simulink model "mainModelDOEJF"  (R2025a)
settings: Solver=VariableStepAuto  StartTime=0  StopTime=1000  RelTol=1e-3
undefined symbols (not defined in the file): advectiveCoefficientScale, AmbientTemperature, coolantTempSourceTemperatureScale, massCoolantScale, massModuleScale, scaledAdvectiveCoefficient, scaledCoolantTemp, scaledMassCoolant, scaledMassModule
libraries: fl_lib x265, nesl_utility x68, coolantFlow_lib x65, thermalCoupledCellResolution_lib x32, heatGenerationForCellResolvedModel x32, batt_lib x1, coolantFlowSwitch_lib x1
(part 3 of 4)

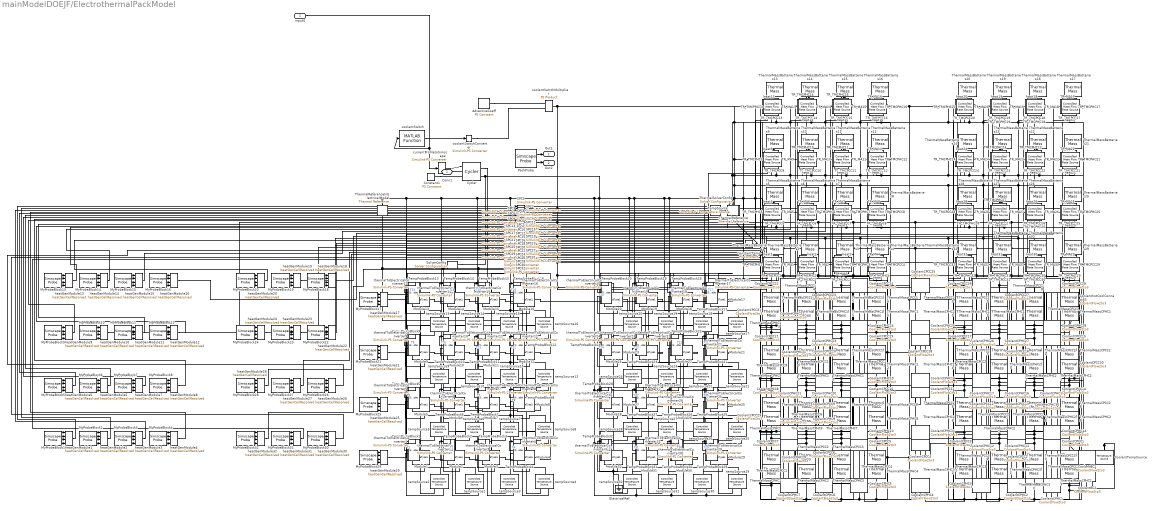
== system mainModelDOEJF/ElectrothermalPackModel ==
  input0 : Inport
  AdvectiveCoeff : fl_lib/Physical Signals/Sources/PS Constant  constant=advectiveCoefficientScale * scaledAdvectiveCoefficient W/K
  Constant1 : fl_lib/Physical Signals/Sources/PS Constant  constant=1
  ConstantTemp : fl_lib/Physical Signals/Sources/PS Constant  constant=AmbientTemperature
  CoolantBC1 : coolantFlow_lib/CoolantFlow2to3  SystemSampleTime=-1  VariantActivationTime=update diagram  EmptyChoice=off  PassThrough=off  PassThroughVariantControl=(default)  EmptyChoiceVariantControl=(default)  AllowFlexibleInterface=on  Latency=0  AutoFrameSizeCalculation=off
  CoolantBC2 : coolantFlow_lib/CoolantFlow2to3  SystemSampleTime=-1  VariantActivationTime=update diagram  EmptyChoice=off  PassThrough=off  PassThroughVariantControl=(default)  EmptyChoiceVariantControl=(default)  AllowFlexibleInterface=on  Latency=0  AutoFrameSizeCalculation=off
  CoolantCPCC{1..31} (31 alike) : coolantFlow_lib/CoolantFlow2to3  SystemSampleTime=-1  VariantActivationTime=update diagram  EmptyChoice=off  PassThrough=off  PassThroughVariantControl=(default)  EmptyChoiceVariantControl=(default)  AllowFlexibleInterface=on  Latency=0  AutoFrameSizeCalculation=off
  CoolantCPHC{1..31} (31 alike) : coolantFlow_lib/CoolantFlow2to3  SystemSampleTime=-1  VariantActivationTime=update diagram  EmptyChoice=off  PassThrough=off  PassThroughVariantControl=(default)  EmptyChoiceVariantControl=(default)  AllowFlexibleInterface=on  Latency=0  AutoFrameSizeCalculation=off
  CoolantTempSource : fl_lib/Thermal/Thermal Sources/Temperature Source  temperature=coolantTempSourceTemperatureScale * scaledCoolantTemp K
  CoolanthotCoolConnect63 : coolantFlow_lib/CoolantFlow2to3  SystemSampleTime=-1  VariantActivationTime=update diagram  EmptyChoice=off  PassThrough=off  PassThroughVariantControl=(default)  EmptyChoiceVariantControl=(default)  AllowFlexibleInterface=on  Latency=0  AutoFrameSizeCalculation=off
  Cycler : batt_lib/Cyclers/Cycler  current_option=simscape.battery.enum.cyclers.positive_current.Discharge  configuration_option=simscape.battery.enum.cyclers.device_configuration.Cycler
      settings: InternalSimscapePortConfiguration="{\"Bottom\":[],\"Left\":[{\"id\":\"iT\",\"label\":\"i\",\"type\":\"input\"},{\"id\":\"vT\",\"label\":\"v\",\"type\":\"input\"},{\"id\":\"c\",\"label\":\"c\",\"type\":\"input\"}],\"Right\":[{\"id\":\"p\",\"label\":\"+\",\"type\":\"foundation.electrical.electrical\"},{\"id\":\"n\",\"label\":\"-\",\"type\":\"foundation.electrical.electrical\"}],\"Top\":[]}"
  ElectricalRef : fl_lib/Electrical/Electrical Elements/Electrical Reference
  Module1 : thermalCoupledCellResolution_lib/Modules/ModuleType1  BatteryCapacityCell=Module01.BatteryCapacityCell A*hr  BatteryCapacityCellPercentDeviation=Module01.BatteryCapacityCellPercentDeviation  ExtrapolationMethodCell=simscape.enum.extrapolation.nearest  SOCBreakpointsCell=Module01.SOCBreakpointsCell  SOCBreakpointsCellPercentDeviation=Module01.SOCBreakpointsCellPercentDeviation  TemperatureBreakpointsCell=Module01.TemperatureBreakpointsCell K  TemperatureBreakpointsCellPercentDeviation=Module01.TemperatureBreakpointsCellPercentDeviation  OpenCircuitVoltageThermalCell=Module01.OpenCircuitVoltageThermalCell V  OpenCircuitVoltageThermalCellPercentDeviation=Module01.OpenCircuitVoltageThermalCellPercentDeviation  VoltageRangeCell=Module01.VoltageRangeCell V  VoltageRangeCellPercentDeviation=Module01.VoltageRangeCellPercentDeviation  ResistanceSOCBreakpointsCell=Module01.ResistanceSOCBreakpointsCell  ResistanceSOCBreakpointsCellPercentDeviation=Module01.ResistanceSOCBreakpointsCellPercentDeviation  ResistanceTemperatureBreakpointsCell=Module01.ResistanceTemperatureBreakpointsCell K  ResistanceTemperatureBreakpointsCellPercentDeviation=Module01.ResistanceTemperatureBreakpointsCellPercentDeviation  R0ThermalCell=Module01.R0ThermalCell Ohm  R0ThermalCellPercentDeviation=Module01.R0ThermalCellPercentDeviation  R1ThermalCell=Module01.R1ThermalCell Ohm  R1ThermalCellPercentDeviation=Module01.R1ThermalCellPercentDeviation  Tau1ThermalCell=Module01.Tau1ThermalCell s  Tau1ThermalCellPercentDeviation=Module01.Tau1ThermalCellPercentDeviation  BatteryThermalMassCell=Module01.BatteryThermalMassCell J/K  BatteryThermalMassCellPercentDeviation=Module01.BatteryThermalMassCellPercentDeviation  AmbientResistance=Module01.AmbientResistance K/W  P=2  S=6  socCell_specify=on  socCell_priority=High  socCell=Module01.socCell  socCell_nominal_specify=off  socCell_nominal_value=1  socCell_nominal_unit=1  batteryVoltage_specify=on  batteryVoltage_priority=None  batteryVoltage=Module01.batteryVoltage V  batteryVoltage_nominal_specify=off  batteryVoltage_nominal_value=1  batteryVoltage_nominal_unit=V  batteryCurrent_specify=on  batteryCurrent_priority=None  batteryCurrent=Module01.batteryCurrent A  batteryCurrent_nominal_specify=off  batteryCurrent_nominal_value=1  batteryCurrent_nominal_unit=A  numCycles_specify=on  numCycles_priority=High  numCycles=Module01.numCycles  numCycles_nominal_specify=off  numCycles_nominal_value=1  numCycles_nominal_unit=1  batteryTemperature_specify=on  batteryTemperature_priority=High  batteryTemperature=Module01.batteryTemperature K  batteryTemperature_nominal_specify=off  batteryTemperature_nominal_value=1  batteryTemperature_nominal_unit=K  vParallelAssembly_specify=on  vParallelAssembly_priority=None  vParallelAssembly=Module01.vParallelAssembly V  vParallelAssembly_nominal_specify=off  vParallelAssembly_nominal_value=1  vParallelAssembly_nominal_unit=V  socParallelAssembly_specify=on  socParallelAssembly_priority=None  socParallelAssembly=Module01.socParallelAssembly  socParallelAssembly_nominal_specify=off  socParallelAssembly_nominal_value=1  socParallelAssembly_nominal_unit=1
      settings: InternalSimscapePortConfiguration="{\"Bottom\":[{\"id\":\"n\",\"label\":\"-\",\"type\":\"foundation.electrical.electrical\"}],\"Left\":[{\"id\":\"AmbH\",\"label\":\"AmbH\",\"type\":\"foundation.thermal.thermal\"}],\"Right\":[],\"Top\":[{\"id\":\"p\",\"label\":\"+\",\"type\":\"foundation.electrical.electrical\"}]}"
  Module10 : thermalCoupledCellResolution_lib/Modules/ModuleType1  BatteryCapacityCell=Module10.BatteryCapacityCell A*hr  BatteryCapacityCellPercentDeviation=Module10.BatteryCapacityCellPercentDeviation  ExtrapolationMethodCell=simscape.enum.extrapolation.nearest  SOCBreakpointsCell=Module10.SOCBreakpointsCell  SOCBreakpointsCellPercentDeviation=Module10.SOCBreakpointsCellPercentDeviation  TemperatureBreakpointsCell=Module10.TemperatureBreakpointsCell K  TemperatureBreakpointsCellPercentDeviation=Module10.TemperatureBreakpointsCellPercentDeviation  OpenCircuitVoltageThermalCell=Module10.OpenCircuitVoltageThermalCell V  OpenCircuitVoltageThermalCellPercentDeviation=Module10.OpenCircuitVoltageThermalCellPercentDeviation  VoltageRangeCell=Module10.VoltageRangeCell V  VoltageRangeCellPercentDeviation=Module10.VoltageRangeCellPercentDeviation  ResistanceSOCBreakpointsCell=Module10.ResistanceSOCBreakpointsCell  ResistanceSOCBreakpointsCellPercentDeviation=Module10.ResistanceSOCBreakpointsCellPercentDeviation  ResistanceTemperatureBreakpointsCell=Module10.ResistanceTemperatureBreakpointsCell K  ResistanceTemperatureBreakpointsCellPercentDeviation=Module10.ResistanceTemperatureBreakpointsCellPercentDeviation  R0ThermalCell=Module10.R0ThermalCell Ohm  R0ThermalCellPercentDeviation=Module10.R0ThermalCellPercentDeviation  R1ThermalCell=Module10.R1ThermalCell Ohm  R1ThermalCellPercentDeviation=Module10.R1ThermalCellPercentDeviation  Tau1ThermalCell=Module10.Tau1ThermalCell s  Tau1ThermalCellPercentDeviation=Module10.Tau1ThermalCellPercentDeviation  BatteryThermalMassCell=Module10.BatteryThermalMassCell J/K  BatteryThermalMassCellPercentDeviation=Module10.BatteryThermalMassCellPercentDeviation  AmbientResistance=Module10.AmbientResistance K/W  P=2  S=6  socCell_specify=on  socCell_priority=High  socCell=Module10.socCell  socCell_nominal_specify=off  socCell_nominal_value=1  socCell_nominal_unit=1  batteryVoltage_specify=on  batteryVoltage_priority=None  batteryVoltage=Module10.batteryVoltage V  batteryVoltage_nominal_specify=off  batteryVoltage_nominal_value=1  batteryVoltage_nominal_unit=V  batteryCurrent_specify=on  batteryCurrent_priority=None  batteryCurrent=Module10.batteryCurrent A  batteryCurrent_nominal_specify=off  batteryCurrent_nominal_value=1  batteryCurrent_nominal_unit=A  numCycles_specify=on  numCycles_priority=High  numCycles=Module10.numCycles  numCycles_nominal_specify=off  numCycles_nominal_value=1  numCycles_nominal_unit=1  batteryTemperature_specify=on  batteryTemperature_priority=High  batteryTemperature=Module10.batteryTemperature K  batteryTemperature_nominal_specify=off  batteryTemperature_nominal_value=1  batteryTemperature_nominal_unit=K  vParallelAssembly_specify=on  vParallelAssembly_priority=None  vParallelAssembly=Module10.vParallelAssembly V  vParallelAssembly_nominal_specify=off  vParallelAssembly_nominal_value=1  vParallelAssembly_nominal_unit=V  socParallelAssembly_specify=on  socParallelAssembly_priority=None  socParallelAssembly=Module10.socParallelAssembly  socParallelAssembly_nominal_specify=off  socParallelAssembly_nominal_value=1  socParallelAssembly_nominal_unit=1
      settings: InternalSimscapePortConfiguration="{\"Bottom\":[{\"id\":\"n\",\"label\":\"-\",\"type\":\"foundation.electrical.electrical\"}],\"Left\":[{\"id\":\"AmbH\",\"label\":\"AmbH\",\"type\":\"foundation.thermal.thermal\"}],\"Right\":[],\"Top\":[{\"id\":\"p\",\"label\":\"+\",\"type\":\"foundation.electrical.electrical\"}]}"
  Module11 : thermalCoupledCellResolution_lib/Modules/ModuleType1  BatteryCapacityCell=Module11.BatteryCapacityCell A*hr  BatteryCapacityCellPercentDeviation=Module11.BatteryCapacityCellPercentDeviation  ExtrapolationMethodCell=simscape.enum.extrapolation.nearest  SOCBreakpointsCell=Module11.SOCBreakpointsCell  SOCBreakpointsCellPercentDeviation=Module11.SOCBreakpointsCellPercentDeviation  TemperatureBreakpointsCell=Module11.TemperatureBreakpointsCell K  TemperatureBreakpointsCellPercentDeviation=Module11.TemperatureBreakpointsCellPercentDeviation  OpenCircuitVoltageThermalCell=Module11.OpenCircuitVoltageThermalCell V  OpenCircuitVoltageThermalCellPercentDeviation=Module11.OpenCircuitVoltageThermalCellPercentDeviation  VoltageRangeCell=Module11.VoltageRangeCell V  VoltageRangeCellPercentDeviation=Module11.VoltageRangeCellPercentDeviation  ResistanceSOCBreakpointsCell=Module11.ResistanceSOCBreakpointsCell  ResistanceSOCBreakpointsCellPercentDeviation=Module11.ResistanceSOCBreakpointsCellPercentDeviation  ResistanceTemperatureBreakpointsCell=Module11.ResistanceTemperatureBreakpointsCell K  ResistanceTemperatureBreakpointsCellPercentDeviation=Module11.ResistanceTemperatureBreakpointsCellPercentDeviation  R0ThermalCell=Module11.R0ThermalCell Ohm  R0ThermalCellPercentDeviation=Module11.R0ThermalCellPercentDeviation  R1ThermalCell=Module11.R1ThermalCell Ohm  R1ThermalCellPercentDeviation=Module11.R1ThermalCellPercentDeviation  Tau1ThermalCell=Module11.Tau1ThermalCell s  Tau1ThermalCellPercentDeviation=Module11.Tau1ThermalCellPercentDeviation  BatteryThermalMassCell=Module11.BatteryThermalMassCell J/K  BatteryThermalMassCellPercentDeviation=Module11.BatteryThermalMassCellPercentDeviation  AmbientResistance=Module11.AmbientResistance K/W  P=2  S=6  socCell_specify=on  socCell_priority=High  socCell=Module11.socCell  socCell_nominal_specify=off  socCell_nominal_value=1  socCell_nominal_unit=1  batteryVoltage_specify=on  batteryVoltage_priority=None  batteryVoltage=Module11.batteryVoltage V  batteryVoltage_nominal_specify=off  batteryVoltage_nominal_value=1  batteryVoltage_nominal_unit=V  batteryCurrent_specify=on  batteryCurrent_priority=None  batteryCurrent=Module11.batteryCurrent A  batteryCurrent_nominal_specify=off  batteryCurrent_nominal_value=1  batteryCurrent_nominal_unit=A  numCycles_specify=on  numCycles_priority=High  numCycles=Module11.numCycles  numCycles_nominal_specify=off  numCycles_nominal_value=1  numCycles_nominal_unit=1  batteryTemperature_specify=on  batteryTemperature_priority=High  batteryTemperature=Module11.batteryTemperature K  batteryTemperature_nominal_specify=off  batteryTemperature_nominal_value=1  batteryTemperature_nominal_unit=K  vParallelAssembly_specify=on  vParallelAssembly_priority=None  vParallelAssembly=Module11.vParallelAssembly V  vParallelAssembly_nominal_specify=off  vParallelAssembly_nominal_value=1  vParallelAssembly_nominal_unit=V  socParallelAssembly_specify=on  socParallelAssembly_priority=None  socParallelAssembly=Module11.socParallelAssembly  socParallelAssembly_nominal_specify=off  socParallelAssembly_nominal_value=1  socParallelAssembly_nominal_unit=1
      settings: InternalSimscapePortConfiguration="{\"Bottom\":[{\"id\":\"n\",\"label\":\"-\",\"type\":\"foundation.electrical.electrical\"}],\"Left\":[{\"id\":\"AmbH\",\"label\":\"AmbH\",\"type\":\"foundation.thermal.thermal\"}],\"Right\":[],\"Top\":[{\"id\":\"p\",\"label\":\"+\",\"type\":\"foundation.electrical.electrical\"}]}"
  Module12 : thermalCoupledCellResolution_lib/Modules/ModuleType1  BatteryCapacityCell=Module12.BatteryCapacityCell A*hr  BatteryCapacityCellPercentDeviation=Module12.BatteryCapacityCellPercentDeviation  ExtrapolationMethodCell=simscape.enum.extrapolation.nearest  SOCBreakpointsCell=Module12.SOCBreakpointsCell  SOCBreakpointsCellPercentDeviation=Module12.SOCBreakpointsCellPercentDeviation  TemperatureBreakpointsCell=Module12.TemperatureBreakpointsCell K  TemperatureBreakpointsCellPercentDeviation=Module12.TemperatureBreakpointsCellPercentDeviation  OpenCircuitVoltageThermalCell=Module12.OpenCircuitVoltageThermalCell V  OpenCircuitVoltageThermalCellPercentDeviation=Module12.OpenCircuitVoltageThermalCellPercentDeviation  VoltageRangeCell=Module12.VoltageRangeCell V  VoltageRangeCellPercentDeviation=Module12.VoltageRangeCellPercentDeviation  ResistanceSOCBreakpointsCell=Module12.ResistanceSOCBreakpointsCell  ResistanceSOCBreakpointsCellPercentDeviation=Module12.ResistanceSOCBreakpointsCellPercentDeviation  ResistanceTemperatureBreakpointsCell=Module12.ResistanceTemperatureBreakpointsCell K  ResistanceTemperatureBreakpointsCellPercentDeviation=Module12.ResistanceTemperatureBreakpointsCellPercentDeviation  R0ThermalCell=Module12.R0ThermalCell Ohm  R0ThermalCellPercentDeviation=Module12.R0ThermalCellPercentDeviation  R1ThermalCell=Module12.R1ThermalCell Ohm  R1ThermalCellPercentDeviation=Module12.R1ThermalCellPercentDeviation  Tau1ThermalCell=Module12.Tau1ThermalCell s  Tau1ThermalCellPercentDeviation=Module12.Tau1ThermalCellPercentDeviation  BatteryThermalMassCell=Module12.BatteryThermalMassCell J/K  BatteryThermalMassCellPercentDeviation=Module12.BatteryThermalMassCellPercentDeviation  AmbientResistance=Module12.AmbientResistance K/W  P=2  S=6  socCell_specify=on  socCell_priority=High  socCell=Module12.socCell  socCell_nominal_specify=off  socCell_nominal_value=1  socCell_nominal_unit=1  batteryVoltage_specify=on  batteryVoltage_priority=None  batteryVoltage=Module12.batteryVoltage V  batteryVoltage_nominal_specify=off  batteryVoltage_nominal_value=1  batteryVoltage_nominal_unit=V  batteryCurrent_specify=on  batteryCurrent_priority=None  batteryCurrent=Module12.batteryCurrent A  batteryCurrent_nominal_specify=off  batteryCurrent_nominal_value=1  batteryCurrent_nominal_unit=A  numCycles_specify=on  numCycles_priority=High  numCycles=Module12.numCycles  numCycles_nominal_specify=off  numCycles_nominal_value=1  numCycles_nominal_unit=1  batteryTemperature_specify=on  batteryTemperature_priority=High  batteryTemperature=Module12.batteryTemperature K  batteryTemperature_nominal_specify=off  batteryTemperature_nominal_value=1  batteryTemperature_nominal_unit=K  vParallelAssembly_specify=on  vParallelAssembly_priority=None  vParallelAssembly=Module12.vParallelAssembly V  vParallelAssembly_nominal_specify=off  vParallelAssembly_nominal_value=1  vParallelAssembly_nominal_unit=V  socParallelAssembly_specify=on  socParallelAssembly_priority=None  socParallelAssembly=Module12.socParallelAssembly  socParallelAssembly_nominal_specify=off  socParallelAssembly_nominal_value=1  socParallelAssembly_nominal_unit=1
      settings: InternalSimscapePortConfiguration="{\"Bottom\":[{\"id\":\"n\",\"label\":\"-\",\"type\":\"foundation.electrical.electrical\"}],\"Left\":[{\"id\":\"AmbH\",\"label\":\"AmbH\",\"type\":\"foundation.thermal.thermal\"}],\"Right\":[],\"Top\":[{\"id\":\"p\",\"label\":\"+\",\"type\":\"foundation.electrical.electrical\"}]}"
  Module13 : thermalCoupledCellResolution_lib/Modules/ModuleType1  BatteryCapacityCell=Module13.BatteryCapacityCell A*hr  BatteryCapacityCellPercentDeviation=Module13.BatteryCapacityCellPercentDeviation  ExtrapolationMethodCell=simscape.enum.extrapolation.nearest  SOCBreakpointsCell=Module13.SOCBreakpointsCell  SOCBreakpointsCellPercentDeviation=Module13.SOCBreakpointsCellPercentDeviation  TemperatureBreakpointsCell=Module13.TemperatureBreakpointsCell K  TemperatureBreakpointsCellPercentDeviation=Module13.TemperatureBreakpointsCellPercentDeviation  OpenCircuitVoltageThermalCell=Module13.OpenCircuitVoltageThermalCell V  OpenCircuitVoltageThermalCellPercentDeviation=Module13.OpenCircuitVoltageThermalCellPercentDeviation  VoltageRangeCell=Module13.VoltageRangeCell V  VoltageRangeCellPercentDeviation=Module13.VoltageRangeCellPercentDeviation  ResistanceSOCBreakpointsCell=Module13.ResistanceSOCBreakpointsCell  ResistanceSOCBreakpointsCellPercentDeviation=Module13.ResistanceSOCBreakpointsCellPercentDeviation  ResistanceTemperatureBreakpointsCell=Module13.ResistanceTemperatureBreakpointsCell K  ResistanceTemperatureBreakpointsCellPercentDeviation=Module13.ResistanceTemperatureBreakpointsCellPercentDeviation  R0ThermalCell=Module13.R0ThermalCell Ohm  R0ThermalCellPercentDeviation=Module13.R0ThermalCellPercentDeviation  R1ThermalCell=Module13.R1ThermalCell Ohm  R1ThermalCellPercentDeviation=Module13.R1ThermalCellPercentDeviation  Tau1ThermalCell=Module13.Tau1ThermalCell s  Tau1ThermalCellPercentDeviation=Module13.Tau1ThermalCellPercentDeviation  BatteryThermalMassCell=Module13.BatteryThermalMassCell J/K  BatteryThermalMassCellPercentDeviation=Module13.BatteryThermalMassCellPercentDeviation  AmbientResistance=Module13.AmbientResistance K/W  P=2  S=6  socCell_specify=on  socCell_priority=High  socCell=Module13.socCell  socCell_nominal_specify=off  socCell_nominal_value=1  socCell_nominal_unit=1  batteryVoltage_specify=on  batteryVoltage_priority=None  batteryVoltage=Module13.batteryVoltage V  batteryVoltage_nominal_specify=off  batteryVoltage_nominal_value=1  batteryVoltage_nominal_unit=V  batteryCurrent_specify=on  batteryCurrent_priority=None  batteryCurrent=Module13.batteryCurrent A  batteryCurrent_nominal_specify=off  batteryCurrent_nominal_value=1  batteryCurrent_nominal_unit=A  numCycles_specify=on  numCycles_priority=High  numCycles=Module13.numCycles  numCycles_nominal_specify=off  numCycles_nominal_value=1  numCycles_nominal_unit=1  batteryTemperature_specify=on  batteryTemperature_priority=High  batteryTemperature=Module13.batteryTemperature K  batteryTemperature_nominal_specify=off  batteryTemperature_nominal_value=1  batteryTemperature_nominal_unit=K  vParallelAssembly_specify=on  vParallelAssembly_priority=None  vParallelAssembly=Module13.vParallelAssembly V  vParallelAssembly_nominal_specify=off  vParallelAssembly_nominal_value=1  vParallelAssembly_nominal_unit=V  socParallelAssembly_specify=on  socParallelAssembly_priority=None  socParallelAssembly=Module13.socParallelAssembly  socParallelAssembly_nominal_specify=off  socParallelAssembly_nominal_value=1  socParallelAssembly_nominal_unit=1
      settings: InternalSimscapePortConfiguration="{\"Bottom\":[{\"id\":\"n\",\"label\":\"-\",\"type\":\"foundation.electrical.electrical\"}],\"Left\":[{\"id\":\"AmbH\",\"label\":\"AmbH\",\"type\":\"foundation.thermal.thermal\"}],\"Right\":[],\"Top\":[{\"id\":\"p\",\"label\":\"+\",\"type\":\"foundation.electrical.electrical\"}]}"
  Module14 : thermalCoupledCellResolution_lib/Modules/ModuleType1  BatteryCapacityCell=Module14.BatteryCapacityCell A*hr  BatteryCapacityCellPercentDeviation=Module14.BatteryCapacityCellPercentDeviation  ExtrapolationMethodCell=simscape.enum.extrapolation.nearest  SOCBreakpointsCell=Module14.SOCBreakpointsCell  SOCBreakpointsCellPercentDeviation=Module14.SOCBreakpointsCellPercentDeviation  TemperatureBreakpointsCell=Module14.TemperatureBreakpointsCell K  TemperatureBreakpointsCellPercentDeviation=Module14.TemperatureBreakpointsCellPercentDeviation  OpenCircuitVoltageThermalCell=Module14.OpenCircuitVoltageThermalCell V  OpenCircuitVoltageThermalCellPercentDeviation=Module14.OpenCircuitVoltageThermalCellPercentDeviation  VoltageRangeCell=Module14.VoltageRangeCell V  VoltageRangeCellPercentDeviation=Module14.VoltageRangeCellPercentDeviation  ResistanceSOCBreakpointsCell=Module14.ResistanceSOCBreakpointsCell  ResistanceSOCBreakpointsCellPercentDeviation=Module14.ResistanceSOCBreakpointsCellPercentDeviation  ResistanceTemperatureBreakpointsCell=Module14.ResistanceTemperatureBreakpointsCell K  ResistanceTemperatureBreakpointsCellPercentDeviation=Module14.ResistanceTemperatureBreakpointsCellPercentDeviation  R0ThermalCell=Module14.R0ThermalCell Ohm  R0ThermalCellPercentDeviation=Module14.R0ThermalCellPercentDeviation  R1ThermalCell=Module14.R1ThermalCell Ohm  R1ThermalCellPercentDeviation=Module14.R1ThermalCellPercentDeviation  Tau1ThermalCell=Module14.Tau1ThermalCell s  Tau1ThermalCellPercentDeviation=Module14.Tau1ThermalCellPercentDeviation  BatteryThermalMassCell=Module14.BatteryThermalMassCell J/K  BatteryThermalMassCellPercentDeviation=Module14.BatteryThermalMassCellPercentDeviation  AmbientResistance=Module14.AmbientResistance K/W  P=2  S=6  socCell_specify=on  socCell_priority=High  socCell=Module14.socCell  socCell_nominal_specify=off  socCell_nominal_value=1  socCell_nominal_unit=1  batteryVoltage_specify=on  batteryVoltage_priority=None  batteryVoltage=Module14.batteryVoltage V  batteryVoltage_nominal_specify=off  batteryVoltage_nominal_value=1  batteryVoltage_nominal_unit=V  batteryCurrent_specify=on  batteryCurrent_priority=None  batteryCurrent=Module14.batteryCurrent A  batteryCurrent_nominal_specify=off  batteryCurrent_nominal_value=1  batteryCurrent_nominal_unit=A  numCycles_specify=on  numCycles_priority=High  numCycles=Module14.numCycles  numCycles_nominal_specify=off  numCycles_nominal_value=1  numCycles_nominal_unit=1  batteryTemperature_specify=on  batteryTemperature_priority=High  batteryTemperature=Module14.batteryTemperature K  batteryTemperature_nominal_specify=off  batteryTemperature_nominal_value=1  batteryTemperature_nominal_unit=K  vParallelAssembly_specify=on  vParallelAssembly_priority=None  vParallelAssembly=Module14.vParallelAssembly V  vParallelAssembly_nominal_specify=off  vParallelAssembly_nominal_value=1  vParallelAssembly_nominal_unit=V  socParallelAssembly_specify=on  socParallelAssembly_priority=None  socParallelAssembly=Module14.socParallelAssembly  socParallelAssembly_nominal_specify=off  socParallelAssembly_nominal_value=1  socParallelAssembly_nominal_unit=1
      settings: InternalSimscapePortConfiguration="{\"Bottom\":[{\"id\":\"n\",\"label\":\"-\",\"type\":\"foundation.electrical.electrical\"}],\"Left\":[{\"id\":\"AmbH\",\"label\":\"AmbH\",\"type\":\"foundation.thermal.thermal\"}],\"Right\":[],\"Top\":[{\"id\":\"p\",\"label\":\"+\",\"type\":\"foundation.electrical.electrical\"}]}"
  Module15 : thermalCoupledCellResolution_lib/Modules/ModuleType1  BatteryCapacityCell=Module15.BatteryCapacityCell A*hr  BatteryCapacityCellPercentDeviation=Module15.BatteryCapacityCellPercentDeviation  ExtrapolationMethodCell=simscape.enum.extrapolation.nearest  SOCBreakpointsCell=Module15.SOCBreakpointsCell  SOCBreakpointsCellPercentDeviation=Module15.SOCBreakpointsCellPercentDeviation  TemperatureBreakpointsCell=Module15.TemperatureBreakpointsCell K  TemperatureBreakpointsCellPercentDeviation=Module15.TemperatureBreakpointsCellPercentDeviation  OpenCircuitVoltageThermalCell=Module15.OpenCircuitVoltageThermalCell V  OpenCircuitVoltageThermalCellPercentDeviation=Module15.OpenCircuitVoltageThermalCellPercentDeviation  VoltageRangeCell=Module15.VoltageRangeCell V  VoltageRangeCellPercentDeviation=Module15.VoltageRangeCellPercentDeviation  ResistanceSOCBreakpointsCell=Module15.ResistanceSOCBreakpointsCell  ResistanceSOCBreakpointsCellPercentDeviation=Module15.ResistanceSOCBreakpointsCellPercentDeviation  ResistanceTemperatureBreakpointsCell=Module15.ResistanceTemperatureBreakpointsCell K  ResistanceTemperatureBreakpointsCellPercentDeviation=Module15.ResistanceTemperatureBreakpointsCellPercentDeviation  R0ThermalCell=Module15.R0ThermalCell Ohm  R0ThermalCellPercentDeviation=Module15.R0ThermalCellPercentDeviation  R1ThermalCell=Module15.R1ThermalCell Ohm  R1ThermalCellPercentDeviation=Module15.R1ThermalCellPercentDeviation  Tau1ThermalCell=Module15.Tau1ThermalCell s  Tau1ThermalCellPercentDeviation=Module15.Tau1ThermalCellPercentDeviation  BatteryThermalMassCell=Module15.BatteryThermalMassCell J/K  BatteryThermalMassCellPercentDeviation=Module15.BatteryThermalMassCellPercentDeviation  AmbientResistance=Module15.AmbientResistance K/W  P=2  S=6  socCell_specify=on  socCell_priority=High  socCell=Module15.socCell  socCell_nominal_specify=off  socCell_nominal_value=1  socCell_nominal_unit=1  batteryVoltage_specify=on  batteryVoltage_priority=None  batteryVoltage=Module15.batteryVoltage V  batteryVoltage_nominal_specify=off  batteryVoltage_nominal_value=1  batteryVoltage_nominal_unit=V  batteryCurrent_specify=on  batteryCurrent_priority=None  batteryCurrent=Module15.batteryCurrent A  batteryCurrent_nominal_specify=off  batteryCurrent_nominal_value=1  batteryCurrent_nominal_unit=A  numCycles_specify=on  numCycles_priority=High  numCycles=Module15.numCycles  numCycles_nominal_specify=off  numCycles_nominal_value=1  numCycles_nominal_unit=1  batteryTemperature_specify=on  batteryTemperature_priority=High  batteryTemperature=Module15.batteryTemperature K  batteryTemperature_nominal_specify=off  batteryTemperature_nominal_value=1  batteryTemperature_nominal_unit=K  vParallelAssembly_specify=on  vParallelAssembly_priority=None  vParallelAssembly=Module15.vParallelAssembly V  vParallelAssembly_nominal_specify=off  vParallelAssembly_nominal_value=1  vParallelAssembly_nominal_unit=V  socParallelAssembly_specify=on  socParallelAssembly_priority=None  socParallelAssembly=Module15.socParallelAssembly  socParallelAssembly_nominal_specify=off  socParallelAssembly_nominal_value=1  socParallelAssembly_nominal_unit=1
      settings: InternalSimscapePortConfiguration="{\"Bottom\":[{\"id\":\"n\",\"label\":\"-\",\"type\":\"foundation.electrical.electrical\"}],\"Left\":[{\"id\":\"AmbH\",\"label\":\"AmbH\",\"type\":\"foundation.thermal.thermal\"}],\"Right\":[],\"Top\":[{\"id\":\"p\",\"label\":\"+\",\"type\":\"foundation.electrical.electrical\"}]}"
  Module16 : thermalCoupledCellResolution_lib/Modules/ModuleType1  BatteryCapacityCell=Module16.BatteryCapacityCell A*hr  BatteryCapacityCellPercentDeviation=Module16.BatteryCapacityCellPercentDeviation  ExtrapolationMethodCell=simscape.enum.extrapolation.nearest  SOCBreakpointsCell=Module16.SOCBreakpointsCell  SOCBreakpointsCellPercentDeviation=Module16.SOCBreakpointsCellPercentDeviation  TemperatureBreakpointsCell=Module16.TemperatureBreakpointsCell K  TemperatureBreakpointsCellPercentDeviation=Module16.TemperatureBreakpointsCellPercentDeviation  OpenCircuitVoltageThermalCell=Module16.OpenCircuitVoltageThermalCell V  OpenCircuitVoltageThermalCellPercentDeviation=Module16.OpenCircuitVoltageThermalCellPercentDeviation  VoltageRangeCell=Module16.VoltageRangeCell V  VoltageRangeCellPercentDeviation=Module16.VoltageRangeCellPercentDeviation  ResistanceSOCBreakpointsCell=Module16.ResistanceSOCBreakpointsCell  ResistanceSOCBreakpointsCellPercentDeviation=Module16.ResistanceSOCBreakpointsCellPercentDeviation  ResistanceTemperatureBreakpointsCell=Module16.ResistanceTemperatureBreakpointsCell K  ResistanceTemperatureBreakpointsCellPercentDeviation=Module16.ResistanceTemperatureBreakpointsCellPercentDeviation  R0ThermalCell=Module16.R0ThermalCell Ohm  R0ThermalCellPercentDeviation=Module16.R0ThermalCellPercentDeviation  R1ThermalCell=Module16.R1ThermalCell Ohm  R1ThermalCellPercentDeviation=Module16.R1ThermalCellPercentDeviation  Tau1ThermalCell=Module16.Tau1ThermalCell s  Tau1ThermalCellPercentDeviation=Module16.Tau1ThermalCellPercentDeviation  BatteryThermalMassCell=Module16.BatteryThermalMassCell J/K  BatteryThermalMassCellPercentDeviation=Module16.BatteryThermalMassCellPercentDeviation  AmbientResistance=Module16.AmbientResistance K/W  P=2  S=6  socCell_specify=on  socCell_priority=High  socCell=Module16.socCell  socCell_nominal_specify=off  socCell_nominal_value=1  socCell_nominal_unit=1  batteryVoltage_specify=on  batteryVoltage_priority=None  batteryVoltage=Module16.batteryVoltage V  batteryVoltage_nominal_specify=off  batteryVoltage_nominal_value=1  batteryVoltage_nominal_unit=V  batteryCurrent_specify=on  batteryCurrent_priority=None  batteryCurrent=Module16.batteryCurrent A  batteryCurrent_nominal_specify=off  batteryCurrent_nominal_value=1  batteryCurrent_nominal_unit=A  numCycles_specify=on  numCycles_priority=High  numCycles=Module16.numCycles  numCycles_nominal_specify=off  numCycles_nominal_value=1  numCycles_nominal_unit=1  batteryTemperature_specify=on  batteryTemperature_priority=High  batteryTemperature=Module16.batteryTemperature K  batteryTemperature_nominal_specify=off  batteryTemperature_nominal_value=1  batteryTemperature_nominal_unit=K  vParallelAssembly_specify=on  vParallelAssembly_priority=None  vParallelAssembly=Module16.vParallelAssembly V  vParallelAssembly_nominal_specify=off  vParallelAssembly_nominal_value=1  vParallelAssembly_nominal_unit=V  socParallelAssembly_specify=on  socParallelAssembly_priority=None  socParallelAssembly=Module16.socParallelAssembly  socParallelAssembly_nominal_specify=off  socParallelAssembly_nominal_value=1  socParallelAssembly_nominal_unit=1
      settings: InternalSimscapePortConfiguration="{\"Bottom\":[{\"id\":\"n\",\"label\":\"-\",\"type\":\"foundation.electrical.electrical\"}],\"Left\":[{\"id\":\"AmbH\",\"label\":\"AmbH\",\"type\":\"foundation.thermal.thermal\"}],\"Right\":[],\"Top\":[{\"id\":\"p\",\"label\":\"+\",\"type\":\"foundation.electrical.electrical\"}]}"
  Module17 : thermalCoupledCellResolution_lib/Modules/ModuleType1  BatteryCapacityCell=Module17.BatteryCapacityCell A*hr  BatteryCapacityCellPercentDeviation=Module17.BatteryCapacityCellPercentDeviation  ExtrapolationMethodCell=simscape.enum.extrapolation.nearest  SOCBreakpointsCell=Module17.SOCBreakpointsCell  SOCBreakpointsCellPercentDeviation=Module17.SOCBreakpointsCellPercentDeviation  TemperatureBreakpointsCell=Module17.TemperatureBreakpointsCell K  TemperatureBreakpointsCellPercentDeviation=Module17.TemperatureBreakpointsCellPercentDeviation  OpenCircuitVoltageThermalCell=Module17.OpenCircuitVoltageThermalCell V  OpenCircuitVoltageThermalCellPercentDeviation=Module17.OpenCircuitVoltageThermalCellPercentDeviation  VoltageRangeCell=Module17.VoltageRangeCell V  VoltageRangeCellPercentDeviation=Module17.VoltageRangeCellPercentDeviation  ResistanceSOCBreakpointsCell=Module17.ResistanceSOCBreakpointsCell  ResistanceSOCBreakpointsCellPercentDeviation=Module17.ResistanceSOCBreakpointsCellPercentDeviation  ResistanceTemperatureBreakpointsCell=Module17.ResistanceTemperatureBreakpointsCell K  ResistanceTemperatureBreakpointsCellPercentDeviation=Module17.ResistanceTemperatureBreakpointsCellPercentDeviation  R0ThermalCell=Module17.R0ThermalCell Ohm  R0ThermalCellPercentDeviation=Module17.R0ThermalCellPercentDeviation  R1ThermalCell=Module17.R1ThermalCell Ohm  R1ThermalCellPercentDeviation=Module17.R1ThermalCellPercentDeviation  Tau1ThermalCell=Module17.Tau1ThermalCell s  Tau1ThermalCellPercentDeviation=Module17.Tau1ThermalCellPercentDeviation  BatteryThermalMassCell=Module17.BatteryThermalMassCell J/K  BatteryThermalMassCellPercentDeviation=Module17.BatteryThermalMassCellPercentDeviation  AmbientResistance=Module17.AmbientResistance K/W  P=2  S=6  socCell_specify=on  socCell_priority=High  socCell=Module17.socCell  socCell_nominal_specify=off  socCell_nominal_value=1  socCell_nominal_unit=1  batteryVoltage_specify=on  batteryVoltage_priority=None  batteryVoltage=Module17.batteryVoltage V  batteryVoltage_nominal_specify=off  batteryVoltage_nominal_value=1  batteryVoltage_nominal_unit=V  batteryCurrent_specify=on  batteryCurrent_priority=None  batteryCurrent=Module17.batteryCurrent A  batteryCurrent_nominal_specify=off  batteryCurrent_nominal_value=1  batteryCurrent_nominal_unit=A  numCycles_specify=on  numCycles_priority=High  numCycles=Module17.numCycles  numCycles_nominal_specify=off  numCycles_nominal_value=1  numCycles_nominal_unit=1  batteryTemperature_specify=on  batteryTemperature_priority=High  batteryTemperature=Module17.batteryTemperature K  batteryTemperature_nominal_specify=off  batteryTemperature_nominal_value=1  batteryTemperature_nominal_unit=K  vParallelAssembly_specify=on  vParallelAssembly_priority=None  vParallelAssembly=Module17.vParallelAssembly V  vParallelAssembly_nominal_specify=off  vParallelAssembly_nominal_value=1  vParallelAssembly_nominal_unit=V  socParallelAssembly_specify=on  socParallelAssembly_priority=None  socParallelAssembly=Module17.socParallelAssembly  socParallelAssembly_nominal_specify=off  socParallelAssembly_nominal_value=1  socParallelAssembly_nominal_unit=1
      settings: InternalSimscapePortConfiguration="{\"Bottom\":[{\"id\":\"n\",\"label\":\"-\",\"type\":\"foundation.electrical.electrical\"}],\"Left\":[{\"id\":\"AmbH\",\"label\":\"AmbH\",\"type\":\"foundation.thermal.thermal\"}],\"Right\":[],\"Top\":[{\"id\":\"p\",\"label\":\"+\",\"type\":\"foundation.electrical.electrical\"}]}"
  Module18 : thermalCoupledCellResolution_lib/Modules/ModuleType1  BatteryCapacityCell=Module18.BatteryCapacityCell A*hr  BatteryCapacityCellPercentDeviation=Module18.BatteryCapacityCellPercentDeviation  ExtrapolationMethodCell=simscape.enum.extrapolation.nearest  SOCBreakpointsCell=Module18.SOCBreakpointsCell  SOCBreakpointsCellPercentDeviation=Module18.SOCBreakpointsCellPercentDeviation  TemperatureBreakpointsCell=Module18.TemperatureBreakpointsCell K  TemperatureBreakpointsCellPercentDeviation=Module18.TemperatureBreakpointsCellPercentDeviation  OpenCircuitVoltageThermalCell=Module18.OpenCircuitVoltageThermalCell V  OpenCircuitVoltageThermalCellPercentDeviation=Module18.OpenCircuitVoltageThermalCellPercentDeviation  VoltageRangeCell=Module18.VoltageRangeCell V  VoltageRangeCellPercentDeviation=Module18.VoltageRangeCellPercentDeviation  ResistanceSOCBreakpointsCell=Module18.ResistanceSOCBreakpointsCell  ResistanceSOCBreakpointsCellPercentDeviation=Module18.ResistanceSOCBreakpointsCellPercentDeviation  ResistanceTemperatureBreakpointsCell=Module18.ResistanceTemperatureBreakpointsCell K  ResistanceTemperatureBreakpointsCellPercentDeviation=Module18.ResistanceTemperatureBreakpointsCellPercentDeviation  R0ThermalCell=Module18.R0ThermalCell Ohm  R0ThermalCellPercentDeviation=Module18.R0ThermalCellPercentDeviation  R1ThermalCell=Module18.R1ThermalCell Ohm  R1ThermalCellPercentDeviation=Module18.R1ThermalCellPercentDeviation  Tau1ThermalCell=Module18.Tau1ThermalCell s  Tau1ThermalCellPercentDeviation=Module18.Tau1ThermalCellPercentDeviation  BatteryThermalMassCell=Module18.BatteryThermalMassCell J/K  BatteryThermalMassCellPercentDeviation=Module18.BatteryThermalMassCellPercentDeviation  AmbientResistance=Module18.AmbientResistance K/W  P=2  S=6  socCell_specify=on  socCell_priority=High  socCell=Module18.socCell  socCell_nominal_specify=off  socCell_nominal_value=1  socCell_nominal_unit=1  batteryVoltage_specify=on  batteryVoltage_priority=None  batteryVoltage=Module18.batteryVoltage V  batteryVoltage_nominal_specify=off  batteryVoltage_nominal_value=1  batteryVoltage_nominal_unit=V  batteryCurrent_specify=on  batteryCurrent_priority=None  batteryCurrent=Module18.batteryCurrent A  batteryCurrent_nominal_specify=off  batteryCurrent_nominal_value=1  batteryCurrent_nominal_unit=A  numCycles_specify=on  numCycles_priority=High  numCycles=Module18.numCycles  numCycles_nominal_specify=off  numCycles_nominal_value=1  numCycles_nominal_unit=1  batteryTemperature_specify=on  batteryTemperature_priority=High  batteryTemperature=Module18.batteryTemperature K  batteryTemperature_nominal_specify=off  batteryTemperature_nominal_value=1  batteryTemperature_nominal_unit=K  vParallelAssembly_specify=on  vParallelAssembly_priority=None  vParallelAssembly=Module18.vParallelAssembly V  vParallelAssembly_nominal_specify=off  vParallelAssembly_nominal_value=1  vParallelAssembly_nominal_unit=V  socParallelAssembly_specify=on  socParallelAssembly_priority=None  socParallelAssembly=Module18.socParallelAssembly  socParallelAssembly_nominal_specify=off  socParallelAssembly_nominal_value=1  socParallelAssembly_nominal_unit=1
      settings: InternalSimscapePortConfiguration="{\"Bottom\":[{\"id\":\"n\",\"label\":\"-\",\"type\":\"foundation.electrical.electrical\"}],\"Left\":[{\"id\":\"AmbH\",\"label\":\"AmbH\",\"type\":\"foundation.thermal.thermal\"}],\"Right\":[],\"Top\":[{\"id\":\"p\",\"label\":\"+\",\"type\":\"foundation.electrical.electrical\"}]}"
  Module19 : thermalCoupledCellResolution_lib/Modules/ModuleType1  BatteryCapacityCell=Module19.BatteryCapacityCell A*hr  BatteryCapacityCellPercentDeviation=Module19.BatteryCapacityCellPercentDeviation  ExtrapolationMethodCell=simscape.enum.extrapolation.nearest  SOCBreakpointsCell=Module19.SOCBreakpointsCell  SOCBreakpointsCellPercentDeviation=Module19.SOCBreakpointsCellPercentDeviation  TemperatureBreakpointsCell=Module19.TemperatureBreakpointsCell K  TemperatureBreakpointsCellPercentDeviation=Module19.TemperatureBreakpointsCellPercentDeviation  OpenCircuitVoltageThermalCell=Module19.OpenCircuitVoltageThermalCell V  OpenCircuitVoltageThermalCellPercentDeviation=Module19.OpenCircuitVoltageThermalCellPercentDeviation  VoltageRangeCell=Module19.VoltageRangeCell V  VoltageRangeCellPercentDeviation=Module19.VoltageRangeCellPercentDeviation  ResistanceSOCBreakpointsCell=Module19.ResistanceSOCBreakpointsCell  ResistanceSOCBreakpointsCellPercentDeviation=Module19.ResistanceSOCBreakpointsCellPercentDeviation  ResistanceTemperatureBreakpointsCell=Module19.ResistanceTemperatureBreakpointsCell K  ResistanceTemperatureBreakpointsCellPercentDeviation=Module19.ResistanceTemperatureBreakpointsCellPercentDeviation  R0ThermalCell=Module19.R0ThermalCell Ohm  R0ThermalCellPercentDeviation=Module19.R0ThermalCellPercentDeviation  R1ThermalCell=Module19.R1ThermalCell Ohm  R1ThermalCellPercentDeviation=Module19.R1ThermalCellPercentDeviation  Tau1ThermalCell=Module19.Tau1ThermalCell s  Tau1ThermalCellPercentDeviation=Module19.Tau1ThermalCellPercentDeviation  BatteryThermalMassCell=Module19.BatteryThermalMassCell J/K  BatteryThermalMassCellPercentDeviation=Module19.BatteryThermalMassCellPercentDeviation  AmbientResistance=Module19.AmbientResistance K/W  P=2  S=6  socCell_specify=on  socCell_priority=High  socCell=Module19.socCell  socCell_nominal_specify=off  socCell_nominal_value=1  socCell_nominal_unit=1  batteryVoltage_specify=on  batteryVoltage_priority=None  batteryVoltage=Module19.batteryVoltage V  batteryVoltage_nominal_specify=off  batteryVoltage_nominal_value=1  batteryVoltage_nominal_unit=V  batteryCurrent_specify=on  batteryCurrent_priority=None  batteryCurrent=Module19.batteryCurrent A  batteryCurrent_nominal_specify=off  batteryCurrent_nominal_value=1  batteryCurrent_nominal_unit=A  numCycles_specify=on  numCycles_priority=High  numCycles=Module19.numCycles  numCycles_nominal_specify=off  numCycles_nominal_value=1  numCycles_nominal_unit=1  batteryTemperature_specify=on  batteryTemperature_priority=High  batteryTemperature=Module19.batteryTemperature K  batteryTemperature_nominal_specify=off  batteryTemperature_nominal_value=1  batteryTemperature_nominal_unit=K  vParallelAssembly_specify=on  vParallelAssembly_priority=None  vParallelAssembly=Module19.vParallelAssembly V  vParallelAssembly_nominal_specify=off  vParallelAssembly_nominal_value=1  vParallelAssembly_nominal_unit=V  socParallelAssembly_specify=on  socParallelAssembly_priority=None  socParallelAssembly=Module19.socParallelAssembly  socParallelAssembly_nominal_specify=off  socParallelAssembly_nominal_value=1  socParallelAssembly_nominal_unit=1
      settings: InternalSimscapePortConfiguration="{\"Bottom\":[{\"id\":\"n\",\"label\":\"-\",\"type\":\"foundation.electrical.electrical\"}],\"Left\":[{\"id\":\"AmbH\",\"label\":\"AmbH\",\"type\":\"foundation.thermal.thermal\"}],\"Right\":[],\"Top\":[{\"id\":\"p\",\"label\":\"+\",\"type\":\"foundation.electrical.electrical\"}]}"
  Module2 : thermalCoupledCellResolution_lib/Modules/ModuleType1  BatteryCapacityCell=Module02.BatteryCapacityCell A*hr  BatteryCapacityCellPercentDeviation=Module02.BatteryCapacityCellPercentDeviation  ExtrapolationMethodCell=simscape.enum.extrapolation.nearest  SOCBreakpointsCell=Module02.SOCBreakpointsCell  SOCBreakpointsCellPercentDeviation=Module02.SOCBreakpointsCellPercentDeviation  TemperatureBreakpointsCell=Module02.TemperatureBreakpointsCell K  TemperatureBreakpointsCellPercentDeviation=Module02.TemperatureBreakpointsCellPercentDeviation  OpenCircuitVoltageThermalCell=Module02.OpenCircuitVoltageThermalCell V  OpenCircuitVoltageThermalCellPercentDeviation=Module02.OpenCircuitVoltageThermalCellPercentDeviation  VoltageRangeCell=Module02.VoltageRangeCell V  VoltageRangeCellPercentDeviation=Module02.VoltageRangeCellPercentDeviation  ResistanceSOCBreakpointsCell=Module02.ResistanceSOCBreakpointsCell  ResistanceSOCBreakpointsCellPercentDeviation=Module02.ResistanceSOCBreakpointsCellPercentDeviation  ResistanceTemperatureBreakpointsCell=Module02.ResistanceTemperatureBreakpointsCell K  ResistanceTemperatureBreakpointsCellPercentDeviation=Module02.ResistanceTemperatureBreakpointsCellPercentDeviation  R0ThermalCell=Module02.R0ThermalCell Ohm  R0ThermalCellPercentDeviation=Module02.R0ThermalCellPercentDeviation  R1ThermalCell=Module02.R1ThermalCell Ohm  R1ThermalCellPercentDeviation=Module02.R1ThermalCellPercentDeviation  Tau1ThermalCell=Module02.Tau1ThermalCell s  Tau1ThermalCellPercentDeviation=Module02.Tau1ThermalCellPercentDeviation  BatteryThermalMassCell=Module02.BatteryThermalMassCell J/K  BatteryThermalMassCellPercentDeviation=Module02.BatteryThermalMassCellPercentDeviation  AmbientResistance=Module02.AmbientResistance K/W  P=2  S=6  socCell_specify=on  socCell_priority=High  socCell=Module02.socCell  socCell_nominal_specify=off  socCell_nominal_value=1  socCell_nominal_unit=1  batteryVoltage_specify=on  batteryVoltage_priority=None  batteryVoltage=Module02.batteryVoltage V  batteryVoltage_nominal_specify=off  batteryVoltage_nominal_value=1  batteryVoltage_nominal_unit=V  batteryCurrent_specify=on  batteryCurrent_priority=None  batteryCurrent=Module02.batteryCurrent A  batteryCurrent_nominal_specify=off  batteryCurrent_nominal_value=1  batteryCurrent_nominal_unit=A  numCycles_specify=on  numCycles_priority=High  numCycles=Module02.numCycles  numCycles_nominal_specify=off  numCycles_nominal_value=1  numCycles_nominal_unit=1  batteryTemperature_specify=on  batteryTemperature_priority=High  batteryTemperature=Module02.batteryTemperature K  batteryTemperature_nominal_specify=off  batteryTemperature_nominal_value=1  batteryTemperature_nominal_unit=K  vParallelAssembly_specify=on  vParallelAssembly_priority=None  vParallelAssembly=Module02.vParallelAssembly V  vParallelAssembly_nominal_specify=off  vParallelAssembly_nominal_value=1  vParallelAssembly_nominal_unit=V  socParallelAssembly_specify=on  socParallelAssembly_priority=None  socParallelAssembly=Module02.socParallelAssembly  socParallelAssembly_nominal_specify=off  socParallelAssembly_nominal_value=1  socParallelAssembly_nominal_unit=1
      settings: InternalSimscapePortConfiguration="{\"Bottom\":[{\"id\":\"n\",\"label\":\"-\",\"type\":\"foundation.electrical.electrical\"}],\"Left\":[{\"id\":\"AmbH\",\"label\":\"AmbH\",\"type\":\"foundation.thermal.thermal\"}],\"Right\":[],\"Top\":[{\"id\":\"p\",\"label\":\"+\",\"type\":\"foundation.electrical.electrical\"}]}"
  Module20 : thermalCoupledCellResolution_lib/Modules/ModuleType1  BatteryCapacityCell=Module20.BatteryCapacityCell A*hr  BatteryCapacityCellPercentDeviation=Module20.BatteryCapacityCellPercentDeviation  ExtrapolationMethodCell=simscape.enum.extrapolation.nearest  SOCBreakpointsCell=Module20.SOCBreakpointsCell  SOCBreakpointsCellPercentDeviation=Module20.SOCBreakpointsCellPercentDeviation  TemperatureBreakpointsCell=Module20.TemperatureBreakpointsCell K  TemperatureBreakpointsCellPercentDeviation=Module20.TemperatureBreakpointsCellPercentDeviation  OpenCircuitVoltageThermalCell=Module20.OpenCircuitVoltageThermalCell V  OpenCircuitVoltageThermalCellPercentDeviation=Module20.OpenCircuitVoltageThermalCellPercentDeviation  VoltageRangeCell=Module20.VoltageRangeCell V  VoltageRangeCellPercentDeviation=Module20.VoltageRangeCellPercentDeviation  ResistanceSOCBreakpointsCell=Module20.ResistanceSOCBreakpointsCell  ResistanceSOCBreakpointsCellPercentDeviation=Module20.ResistanceSOCBreakpointsCellPercentDeviation  ResistanceTemperatureBreakpointsCell=Module20.ResistanceTemperatureBreakpointsCell K  ResistanceTemperatureBreakpointsCellPercentDeviation=Module20.ResistanceTemperatureBreakpointsCellPercentDeviation  R0ThermalCell=Module20.R0ThermalCell Ohm  R0ThermalCellPercentDeviation=Module20.R0ThermalCellPercentDeviation  R1ThermalCell=Module20.R1ThermalCell Ohm  R1ThermalCellPercentDeviation=Module20.R1ThermalCellPercentDeviation  Tau1ThermalCell=Module20.Tau1ThermalCell s  Tau1ThermalCellPercentDeviation=Module20.Tau1ThermalCellPercentDeviation  BatteryThermalMassCell=Module20.BatteryThermalMassCell J/K  BatteryThermalMassCellPercentDeviation=Module20.BatteryThermalMassCellPercentDeviation  AmbientResistance=Module20.AmbientResistance K/W  P=2  S=6  socCell_specify=on  socCell_priority=High  socCell=Module20.socCell  socCell_nominal_specify=off  socCell_nominal_value=1  socCell_nominal_unit=1  batteryVoltage_specify=on  batteryVoltage_priority=None  batteryVoltage=Module20.batteryVoltage V  batteryVoltage_nominal_specify=off  batteryVoltage_nominal_value=1  batteryVoltage_nominal_unit=V  batteryCurrent_specify=on  batteryCurrent_priority=None  batteryCurrent=Module20.batteryCurrent A  batteryCurrent_nominal_specify=off  batteryCurrent_nominal_value=1  batteryCurrent_nominal_unit=A  numCycles_specify=on  numCycles_priority=High  numCycles=Module20.numCycles  numCycles_nominal_specify=off  numCycles_nominal_value=1  numCycles_nominal_unit=1  batteryTemperature_specify=on  batteryTemperature_priority=High  batteryTemperature=Module20.batteryTemperature K  batteryTemperature_nominal_specify=off  batteryTemperature_nominal_value=1  batteryTemperature_nominal_unit=K  vParallelAssembly_specify=on  vParallelAssembly_priority=None  vParallelAssembly=Module20.vParallelAssembly V  vParallelAssembly_nominal_specify=off  vParallelAssembly_nominal_value=1  vParallelAssembly_nominal_unit=V  socParallelAssembly_specify=on  socParallelAssembly_priority=None  socParallelAssembly=Module20.socParallelAssembly  socParallelAssembly_nominal_specify=off  socParallelAssembly_nominal_value=1  socParallelAssembly_nominal_unit=1
      settings: InternalSimscapePortConfiguration="{\"Bottom\":[{\"id\":\"n\",\"label\":\"-\",\"type\":\"foundation.electrical.electrical\"}],\"Left\":[{\"id\":\"AmbH\",\"label\":\"AmbH\",\"type\":\"foundation.thermal.thermal\"}],\"Right\":[],\"Top\":[{\"id\":\"p\",\"label\":\"+\",\"type\":\"foundation.electrical.electrical\"}]}"
  Module21 : thermalCoupledCellResolution_lib/Modules/ModuleType1  BatteryCapacityCell=Module21.BatteryCapacityCell A*hr  BatteryCapacityCellPercentDeviation=Module21.BatteryCapacityCellPercentDeviation  ExtrapolationMethodCell=simscape.enum.extrapolation.nearest  SOCBreakpointsCell=Module21.SOCBreakpointsCell  SOCBreakpointsCellPercentDeviation=Module21.SOCBreakpointsCellPercentDeviation  TemperatureBreakpointsCell=Module21.TemperatureBreakpointsCell K  TemperatureBreakpointsCellPercentDeviation=Module21.TemperatureBreakpointsCellPercentDeviation  OpenCircuitVoltageThermalCell=Module21.OpenCircuitVoltageThermalCell V  OpenCircuitVoltageThermalCellPercentDeviation=Module21.OpenCircuitVoltageThermalCellPercentDeviation  VoltageRangeCell=Module21.VoltageRangeCell V  VoltageRangeCellPercentDeviation=Module21.VoltageRangeCellPercentDeviation  ResistanceSOCBreakpointsCell=Module21.ResistanceSOCBreakpointsCell  ResistanceSOCBreakpointsCellPercentDeviation=Module21.ResistanceSOCBreakpointsCellPercentDeviation  ResistanceTemperatureBreakpointsCell=Module21.ResistanceTemperatureBreakpointsCell K  ResistanceTemperatureBreakpointsCellPercentDeviation=Module21.ResistanceTemperatureBreakpointsCellPercentDeviation  R0ThermalCell=Module21.R0ThermalCell Ohm  R0ThermalCellPercentDeviation=Module21.R0ThermalCellPercentDeviation  R1ThermalCell=Module21.R1ThermalCell Ohm  R1ThermalCellPercentDeviation=Module21.R1ThermalCellPercentDeviation  Tau1ThermalCell=Module21.Tau1ThermalCell s  Tau1ThermalCellPercentDeviation=Module21.Tau1ThermalCellPercentDeviation  BatteryThermalMassCell=Module21.BatteryThermalMassCell J/K  BatteryThermalMassCellPercentDeviation=Module21.BatteryThermalMassCellPercentDeviation  AmbientResistance=Module21.AmbientResistance K/W  P=2  S=6  socCell_specify=on  socCell_priority=High  socCell=Module21.socCell  socCell_nominal_specify=off  socCell_nominal_value=1  socCell_nominal_unit=1  batteryVoltage_specify=on  batteryVoltage_priority=None  batteryVoltage=Module21.batteryVoltage V  batteryVoltage_nominal_specify=off  batteryVoltage_nominal_value=1  batteryVoltage_nominal_unit=V  batteryCurrent_specify=on  batteryCurrent_priority=None  batteryCurrent=Module21.batteryCurrent A  batteryCurrent_nominal_specify=off  batteryCurrent_nominal_value=1  batteryCurrent_nominal_unit=A  numCycles_specify=on  numCycles_priority=High  numCycles=Module21.numCycles  numCycles_nominal_specify=off  numCycles_nominal_value=1  numCycles_nominal_unit=1  batteryTemperature_specify=on  batteryTemperature_priority=High  batteryTemperature=Module21.batteryTemperature K  batteryTemperature_nominal_specify=off  batteryTemperature_nominal_value=1  batteryTemperature_nominal_unit=K  vParallelAssembly_specify=on  vParallelAssembly_priority=None  vParallelAssembly=Module21.vParallelAssembly V  vParallelAssembly_nominal_specify=off  vParallelAssembly_nominal_value=1  vParallelAssembly_nominal_unit=V  socParallelAssembly_specify=on  socParallelAssembly_priority=None  socParallelAssembly=Module21.socParallelAssembly  socParallelAssembly_nominal_specify=off  socParallelAssembly_nominal_value=1  socParallelAssembly_nominal_unit=1
      settings: InternalSimscapePortConfiguration="{\"Bottom\":[{\"id\":\"n\",\"label\":\"-\",\"type\":\"foundation.electrical.electrical\"}],\"Left\":[{\"id\":\"AmbH\",\"label\":\"AmbH\",\"type\":\"foundation.thermal.thermal\"}],\"Right\":[],\"Top\":[{\"id\":\"p\",\"label\":\"+\",\"type\":\"foundation.electrical.electrical\"}]}"
  Module22 : thermalCoupledCellResolution_lib/Modules/ModuleType1  BatteryCapacityCell=Module22.BatteryCapacityCell A*hr  BatteryCapacityCellPercentDeviation=Module22.BatteryCapacityCellPercentDeviation  ExtrapolationMethodCell=simscape.enum.extrapolation.nearest  SOCBreakpointsCell=Module22.SOCBreakpointsCell  SOCBreakpointsCellPercentDeviation=Module22.SOCBreakpointsCellPercentDeviation  TemperatureBreakpointsCell=Module22.TemperatureBreakpointsCell K  TemperatureBreakpointsCellPercentDeviation=Module22.TemperatureBreakpointsCellPercentDeviation  OpenCircuitVoltageThermalCell=Module22.OpenCircuitVoltageThermalCell V  OpenCircuitVoltageThermalCellPercentDeviation=Module22.OpenCircuitVoltageThermalCellPercentDeviation  VoltageRangeCell=Module22.VoltageRangeCell V  VoltageRangeCellPercentDeviation=Module22.VoltageRangeCellPercentDeviation  ResistanceSOCBreakpointsCell=Module22.ResistanceSOCBreakpointsCell  ResistanceSOCBreakpointsCellPercentDeviation=Module22.ResistanceSOCBreakpointsCellPercentDeviation  ResistanceTemperatureBreakpointsCell=Module22.ResistanceTemperatureBreakpointsCell K  ResistanceTemperatureBreakpointsCellPercentDeviation=Module22.ResistanceTemperatureBreakpointsCellPercentDeviation  R0ThermalCell=Module22.R0ThermalCell Ohm  R0ThermalCellPercentDeviation=Module22.R0ThermalCellPercentDeviation  R1ThermalCell=Module22.R1ThermalCell Ohm  R1ThermalCellPercentDeviation=Module22.R1ThermalCellPercentDeviation  Tau1ThermalCell=Module22.Tau1ThermalCell s  Tau1ThermalCellPercentDeviation=Module22.Tau1ThermalCellPercentDeviation  BatteryThermalMassCell=Module22.BatteryThermalMassCell J/K  BatteryThermalMassCellPercentDeviation=Module22.BatteryThermalMassCellPercentDeviation  AmbientResistance=Module22.AmbientResistance K/W  P=2  S=6  socCell_specify=on  socCell_priority=High  socCell=Module22.socCell  socCell_nominal_specify=off  socCell_nominal_value=1  socCell_nominal_unit=1  batteryVoltage_specify=on  batteryVoltage_priority=None  batteryVoltage=Module22.batteryVoltage V  batteryVoltage_nominal_specify=off  batteryVoltage_nominal_value=1  batteryVoltage_nominal_unit=V  batteryCurrent_specify=on  batteryCurrent_priority=None  batteryCurrent=Module22.batteryCurrent A  batteryCurrent_nominal_specify=off  batteryCurrent_nominal_value=1  batteryCurrent_nominal_unit=A  numCycles_specify=on  numCycles_priority=High  numCycles=Module22.numCycles  numCycles_nominal_specify=off  numCycles_nominal_value=1  numCycles_nominal_unit=1  batteryTemperature_specify=on  batteryTemperature_priority=High  batteryTemperature=Module22.batteryTemperature K  batteryTemperature_nominal_specify=off  batteryTemperature_nominal_value=1  batteryTemperature_nominal_unit=K  vParallelAssembly_specify=on  vParallelAssembly_priority=None  vParallelAssembly=Module22.vParallelAssembly V  vParallelAssembly_nominal_specify=off  vParallelAssembly_nominal_value=1  vParallelAssembly_nominal_unit=V  socParallelAssembly_specify=on  socParallelAssembly_priority=None  socParallelAssembly=Module22.socParallelAssembly  socParallelAssembly_nominal_specify=off  socParallelAssembly_nominal_value=1  socParallelAssembly_nominal_unit=1
      settings: InternalSimscapePortConfiguration="{\"Bottom\":[{\"id\":\"n\",\"label\":\"-\",\"type\":\"foundation.electrical.electrical\"}],\"Left\":[{\"id\":\"AmbH\",\"label\":\"AmbH\",\"type\":\"foundation.thermal.thermal\"}],\"Right\":[],\"Top\":[{\"id\":\"p\",\"label\":\"+\",\"type\":\"foundation.electrical.electrical\"}]}"
  Module23 : thermalCoupledCellResolution_lib/Modules/ModuleType1  BatteryCapacityCell=Module23.BatteryCapacityCell A*hr  BatteryCapacityCellPercentDeviation=Module23.BatteryCapacityCellPercentDeviation  ExtrapolationMethodCell=simscape.enum.extrapolation.nearest  SOCBreakpointsCell=Module23.SOCBreakpointsCell  SOCBreakpointsCellPercentDeviation=Module23.SOCBreakpointsCellPercentDeviation  TemperatureBreakpointsCell=Module23.TemperatureBreakpointsCell K  TemperatureBreakpointsCellPercentDeviation=Module23.TemperatureBreakpointsCellPercentDeviation  OpenCircuitVoltageThermalCell=Module23.OpenCircuitVoltageThermalCell V  OpenCircuitVoltageThermalCellPercentDeviation=Module23.OpenCircuitVoltageThermalCellPercentDeviation  VoltageRangeCell=Module23.VoltageRangeCell V  VoltageRangeCellPercentDeviation=Module23.VoltageRangeCellPercentDeviation  ResistanceSOCBreakpointsCell=Module23.ResistanceSOCBreakpointsCell  ResistanceSOCBreakpointsCellPercentDeviation=Module23.ResistanceSOCBreakpointsCellPercentDeviation  ResistanceTemperatureBreakpointsCell=Module23.ResistanceTemperatureBreakpointsCell K  ResistanceTemperatureBreakpointsCellPercentDeviation=Module23.ResistanceTemperatureBreakpointsCellPercentDeviation  R0ThermalCell=Module23.R0ThermalCell Ohm  R0ThermalCellPercentDeviation=Module23.R0ThermalCellPercentDeviation  R1ThermalCell=Module23.R1ThermalCell Ohm  R1ThermalCellPercentDeviation=Module23.R1ThermalCellPercentDeviation  Tau1ThermalCell=Module23.Tau1ThermalCell s  Tau1ThermalCellPercentDeviation=Module23.Tau1ThermalCellPercentDeviation  BatteryThermalMassCell=Module23.BatteryThermalMassCell J/K  BatteryThermalMassCellPercentDeviation=Module23.BatteryThermalMassCellPercentDeviation  AmbientResistance=Module23.AmbientResistance K/W  P=2  S=6  socCell_specify=on  socCell_priority=High  socCell=Module23.socCell  socCell_nominal_specify=off  socCell_nominal_value=1  socCell_nominal_unit=1  batteryVoltage_specify=on  batteryVoltage_priority=None  batteryVoltage=Module23.batteryVoltage V  batteryVoltage_nominal_specify=off  batteryVoltage_nominal_value=1  batteryVoltage_nominal_unit=V  batteryCurrent_specify=on  batteryCurrent_priority=None  batteryCurrent=Module23.batteryCurrent A  batteryCurrent_nominal_specify=off  batteryCurrent_nominal_value=1  batteryCurrent_nominal_unit=A  numCycles_specify=on  numCycles_priority=High  numCycles=Module23.numCycles  numCycles_nominal_specify=off  numCycles_nominal_value=1  numCycles_nominal_unit=1  batteryTemperature_specify=on  batteryTemperature_priority=High  batteryTemperature=Module23.batteryTemperature K  batteryTemperature_nominal_specify=off  batteryTemperature_nominal_value=1  batteryTemperature_nominal_unit=K  vParallelAssembly_specify=on  vParallelAssembly_priority=None  vParallelAssembly=Module23.vParallelAssembly V  vParallelAssembly_nominal_specify=off  vParallelAssembly_nominal_value=1  vParallelAssembly_nominal_unit=V  socParallelAssembly_specify=on  socParallelAssembly_priority=None  socParallelAssembly=Module23.socParallelAssembly  socParallelAssembly_nominal_specify=off  socParallelAssembly_nominal_value=1  socParallelAssembly_nominal_unit=1
      settings: InternalSimscapePortConfiguration="{\"Bottom\":[{\"id\":\"n\",\"label\":\"-\",\"type\":\"foundation.electrical.electrical\"}],\"Left\":[{\"id\":\"AmbH\",\"label\":\"AmbH\",\"type\":\"foundation.thermal.thermal\"}],\"Right\":[],\"Top\":[{\"id\":\"p\",\"label\":\"+\",\"type\":\"foundation.electrical.electrical\"}]}"
  Module24 : thermalCoupledCellResolution_lib/Modules/ModuleType1  BatteryCapacityCell=Module24.BatteryCapacityCell A*hr  BatteryCapacityCellPercentDeviation=Module24.BatteryCapacityCellPercentDeviation  ExtrapolationMethodCell=simscape.enum.extrapolation.nearest  SOCBreakpointsCell=Module24.SOCBreakpointsCell  SOCBreakpointsCellPercentDeviation=Module24.SOCBreakpointsCellPercentDeviation  TemperatureBreakpointsCell=Module24.TemperatureBreakpointsCell K  TemperatureBreakpointsCellPercentDeviation=Module24.TemperatureBreakpointsCellPercentDeviation  OpenCircuitVoltageThermalCell=Module24.OpenCircuitVoltageThermalCell V  OpenCircuitVoltageThermalCellPercentDeviation=Module24.OpenCircuitVoltageThermalCellPercentDeviation  VoltageRangeCell=Module24.VoltageRangeCell V  VoltageRangeCellPercentDeviation=Module24.VoltageRangeCellPercentDeviation  ResistanceSOCBreakpointsCell=Module24.ResistanceSOCBreakpointsCell  ResistanceSOCBreakpointsCellPercentDeviation=Module24.ResistanceSOCBreakpointsCellPercentDeviation  ResistanceTemperatureBreakpointsCell=Module24.ResistanceTemperatureBreakpointsCell K  ResistanceTemperatureBreakpointsCellPercentDeviation=Module24.ResistanceTemperatureBreakpointsCellPercentDeviation  R0ThermalCell=Module24.R0ThermalCell Ohm  R0ThermalCellPercentDeviation=Module24.R0ThermalCellPercentDeviation  R1ThermalCell=Module24.R1ThermalCell Ohm  R1ThermalCellPercentDeviation=Module24.R1ThermalCellPercentDeviation  Tau1ThermalCell=Module24.Tau1ThermalCell s  Tau1ThermalCellPercentDeviation=Module24.Tau1ThermalCellPercentDeviation  BatteryThermalMassCell=Module24.BatteryThermalMassCell J/K  BatteryThermalMassCellPercentDeviation=Module24.BatteryThermalMassCellPercentDeviation  AmbientResistance=Module24.AmbientResistance K/W  P=2  S=6  socCell_specify=on  socCell_priority=High  socCell=Module24.socCell  socCell_nominal_specify=off  socCell_nominal_value=1  socCell_nominal_unit=1  batteryVoltage_specify=on  batteryVoltage_priority=None  batteryVoltage=Module24.batteryVoltage V  batteryVoltage_nominal_specify=off  batteryVoltage_nominal_value=1  batteryVoltage_nominal_unit=V  batteryCurrent_specify=on  batteryCurrent_priority=None  batteryCurrent=Module24.batteryCurrent A  batteryCurrent_nominal_specify=off  batteryCurrent_nominal_value=1  batteryCurrent_nominal_unit=A  numCycles_specify=on  numCycles_priority=High  numCycles=Module24.numCycles  numCycles_nominal_specify=off  numCycles_nominal_value=1  numCycles_nominal_unit=1  batteryTemperature_specify=on  batteryTemperature_priority=High  batteryTemperature=Module24.batteryTemperature K  batteryTemperature_nominal_specify=off  batteryTemperature_nominal_value=1  batteryTemperature_nominal_unit=K  vParallelAssembly_specify=on  vParallelAssembly_priority=None  vParallelAssembly=Module24.vParallelAssembly V  vParallelAssembly_nominal_specify=off  vParallelAssembly_nominal_value=1  vParallelAssembly_nominal_unit=V  socParallelAssembly_specify=on  socParallelAssembly_priority=None  socParallelAssembly=Module24.socParallelAssembly  socParallelAssembly_nominal_specify=off  socParallelAssembly_nominal_value=1  socParallelAssembly_nominal_unit=1
      settings: InternalSimscapePortConfiguration="{\"Bottom\":[{\"id\":\"n\",\"label\":\"-\",\"type\":\"foundation.electrical.electrical\"}],\"Left\":[{\"id\":\"AmbH\",\"label\":\"AmbH\",\"type\":\"foundation.thermal.thermal\"}],\"Right\":[],\"Top\":[{\"id\":\"p\",\"label\":\"+\",\"type\":\"foundation.electrical.electrical\"}]}"
  Module25 : thermalCoupledCellResolution_lib/Modules/ModuleType1  BatteryCapacityCell=Module25.BatteryCapacityCell A*hr  BatteryCapacityCellPercentDeviation=Module25.BatteryCapacityCellPercentDeviation  ExtrapolationMethodCell=simscape.enum.extrapolation.nearest  SOCBreakpointsCell=Module25.SOCBreakpointsCell  SOCBreakpointsCellPercentDeviation=Module25.SOCBreakpointsCellPercentDeviation  TemperatureBreakpointsCell=Module25.TemperatureBreakpointsCell K  TemperatureBreakpointsCellPercentDeviation=Module25.TemperatureBreakpointsCellPercentDeviation  OpenCircuitVoltageThermalCell=Module25.OpenCircuitVoltageThermalCell V  OpenCircuitVoltageThermalCellPercentDeviation=Module25.OpenCircuitVoltageThermalCellPercentDeviation  VoltageRangeCell=Module25.VoltageRangeCell V  VoltageRangeCellPercentDeviation=Module25.VoltageRangeCellPercentDeviation  ResistanceSOCBreakpointsCell=Module25.ResistanceSOCBreakpointsCell  ResistanceSOCBreakpointsCellPercentDeviation=Module25.ResistanceSOCBreakpointsCellPercentDeviation  ResistanceTemperatureBreakpointsCell=Module25.ResistanceTemperatureBreakpointsCell K  ResistanceTemperatureBreakpointsCellPercentDeviation=Module25.ResistanceTemperatureBreakpointsCellPercentDeviation  R0ThermalCell=Module25.R0ThermalCell Ohm  R0ThermalCellPercentDeviation=Module25.R0ThermalCellPercentDeviation  R1ThermalCell=Module25.R1ThermalCell Ohm  R1ThermalCellPercentDeviation=Module25.R1ThermalCellPercentDeviation  Tau1ThermalCell=Module25.Tau1ThermalCell s  Tau1ThermalCellPercentDeviation=Module25.Tau1ThermalCellPercentDeviation  BatteryThermalMassCell=Module25.BatteryThermalMassCell J/K  BatteryThermalMassCellPercentDeviation=Module25.BatteryThermalMassCellPercentDeviation  AmbientResistance=Module25.AmbientResistance K/W  P=2  S=6  socCell_specify=on  socCell_priority=High  socCell=Module25.socCell  socCell_nominal_specify=off  socCell_nominal_value=1  socCell_nominal_unit=1  batteryVoltage_specify=on  batteryVoltage_priority=None  batteryVoltage=Module25.batteryVoltage V  batteryVoltage_nominal_specify=off  batteryVoltage_nominal_value=1  batteryVoltage_nominal_unit=V  batteryCurrent_specify=on  batteryCurrent_priority=None  batteryCurrent=Module25.batteryCurrent A  batteryCurrent_nominal_specify=off  batteryCurrent_nominal_value=1  batteryCurrent_nominal_unit=A  numCycles_specify=on  numCycles_priority=High  numCycles=Module25.numCycles  numCycles_nominal_specify=off  numCycles_nominal_value=1  numCycles_nominal_unit=1  batteryTemperature_specify=on  batteryTemperature_priority=High  batteryTemperature=Module25.batteryTemperature K  batteryTemperature_nominal_specify=off  batteryTemperature_nominal_value=1  batteryTemperature_nominal_unit=K  vParallelAssembly_specify=on  vParallelAssembly_priority=None  vParallelAssembly=Module25.vParallelAssembly V  vParallelAssembly_nominal_specify=off  vParallelAssembly_nominal_value=1  vParallelAssembly_nominal_unit=V  socParallelAssembly_specify=on  socParallelAssembly_priority=None  socParallelAssembly=Module25.socParallelAssembly  socParallelAssembly_nominal_specify=off  socParallelAssembly_nominal_value=1  socParallelAssembly_nominal_unit=1
      settings: InternalSimscapePortConfiguration="{\"Bottom\":[{\"id\":\"n\",\"label\":\"-\",\"type\":\"foundation.electrical.electrical\"}],\"Left\":[{\"id\":\"AmbH\",\"label\":\"AmbH\",\"type\":\"foundation.thermal.thermal\"}],\"Right\":[],\"Top\":[{\"id\":\"p\",\"label\":\"+\",\"type\":\"foundation.electrical.electrical\"}]}"
  Module26 : thermalCoupledCellResolution_lib/Modules/ModuleType1  BatteryCapacityCell=Module26.BatteryCapacityCell A*hr  BatteryCapacityCellPercentDeviation=Module26.BatteryCapacityCellPercentDeviation  ExtrapolationMethodCell=simscape.enum.extrapolation.nearest  SOCBreakpointsCell=Module26.SOCBreakpointsCell  SOCBreakpointsCellPercentDeviation=Module26.SOCBreakpointsCellPercentDeviation  TemperatureBreakpointsCell=Module26.TemperatureBreakpointsCell K  TemperatureBreakpointsCellPercentDeviation=Module26.TemperatureBreakpointsCellPercentDeviation  OpenCircuitVoltageThermalCell=Module26.OpenCircuitVoltageThermalCell V  OpenCircuitVoltageThermalCellPercentDeviation=Module26.OpenCircuitVoltageThermalCellPercentDeviation  VoltageRangeCell=Module26.VoltageRangeCell V  VoltageRangeCellPercentDeviation=Module26.VoltageRangeCellPercentDeviation  ResistanceSOCBreakpointsCell=Module26.ResistanceSOCBreakpointsCell  ResistanceSOCBreakpointsCellPercentDeviation=Module26.ResistanceSOCBreakpointsCellPercentDeviation  ResistanceTemperatureBreakpointsCell=Module26.ResistanceTemperatureBreakpointsCell K  ResistanceTemperatureBreakpointsCellPercentDeviation=Module26.ResistanceTemperatureBreakpointsCellPercentDeviation  R0ThermalCell=Module26.R0ThermalCell Ohm  R0ThermalCellPercentDeviation=Module26.R0ThermalCellPercentDeviation  R1ThermalCell=Module26.R1ThermalCell Ohm  R1ThermalCellPercentDeviation=Module26.R1ThermalCellPercentDeviation  Tau1ThermalCell=Module26.Tau1ThermalCell s  Tau1ThermalCellPercentDeviation=Module26.Tau1ThermalCellPercentDeviation  BatteryThermalMassCell=Module26.BatteryThermalMassCell J/K  BatteryThermalMassCellPercentDeviation=Module26.BatteryThermalMassCellPercentDeviation  AmbientResistance=Module26.AmbientResistance K/W  P=2  S=6  socCell_specify=on  socCell_priority=High  socCell=Module26.socCell  socCell_nominal_specify=off  socCell_nominal_value=1  socCell_nominal_unit=1  batteryVoltage_specify=on  batteryVoltage_priority=None  batteryVoltage=Module26.batteryVoltage V  batteryVoltage_nominal_specify=off  batteryVoltage_nominal_value=1  batteryVoltage_nominal_unit=V  batteryCurrent_specify=on  batteryCurrent_priority=None  batteryCurrent=Module26.batteryCurrent A  batteryCurrent_nominal_specify=off  batteryCurrent_nominal_value=1  batteryCurrent_nominal_unit=A  numCycles_specify=on  numCycles_priority=High  numCycles=Module26.numCycles  numCycles_nominal_specify=off  numCycles_nominal_value=1  numCycles_nominal_unit=1  batteryTemperature_specify=on  batteryTemperature_priority=High  batteryTemperature=Module26.batteryTemperature K  batteryTemperature_nominal_specify=off  batteryTemperature_nominal_value=1  batteryTemperature_nominal_unit=K  vParallelAssembly_specify=on  vParallelAssembly_priority=None  vParallelAssembly=Module26.vParallelAssembly V  vParallelAssembly_nominal_specify=off  vParallelAssembly_nominal_value=1  vParallelAssembly_nominal_unit=V  socParallelAssembly_specify=on  socParallelAssembly_priority=None  socParallelAssembly=Module26.socParallelAssembly  socParallelAssembly_nominal_specify=off  socParallelAssembly_nominal_value=1  socParallelAssembly_nominal_unit=1
      settings: InternalSimscapePortConfiguration="{\"Bottom\":[{\"id\":\"n\",\"label\":\"-\",\"type\":\"foundation.electrical.electrical\"}],\"Left\":[{\"id\":\"AmbH\",\"label\":\"AmbH\",\"type\":\"foundation.thermal.thermal\"}],\"Right\":[],\"Top\":[{\"id\":\"p\",\"label\":\"+\",\"type\":\"foundation.electrical.electrical\"}]}"
  Module27 : thermalCoupledCellResolution_lib/Modules/ModuleType1  BatteryCapacityCell=Module27.BatteryCapacityCell A*hr  BatteryCapacityCellPercentDeviation=Module27.BatteryCapacityCellPercentDeviation  ExtrapolationMethodCell=simscape.enum.extrapolation.nearest  SOCBreakpointsCell=Module27.SOCBreakpointsCell  SOCBreakpointsCellPercentDeviation=Module27.SOCBreakpointsCellPercentDeviation  TemperatureBreakpointsCell=Module27.TemperatureBreakpointsCell K  TemperatureBreakpointsCellPercentDeviation=Module27.TemperatureBreakpointsCellPercentDeviation  OpenCircuitVoltageThermalCell=Module27.OpenCircuitVoltageThermalCell V  OpenCircuitVoltageThermalCellPercentDeviation=Module27.OpenCircuitVoltageThermalCellPercentDeviation  VoltageRangeCell=Module27.VoltageRangeCell V  VoltageRangeCellPercentDeviation=Module27.VoltageRangeCellPercentDeviation  ResistanceSOCBreakpointsCell=Module27.ResistanceSOCBreakpointsCell  ResistanceSOCBreakpointsCellPercentDeviation=Module27.ResistanceSOCBreakpointsCellPercentDeviation  ResistanceTemperatureBreakpointsCell=Module27.ResistanceTemperatureBreakpointsCell K  ResistanceTemperatureBreakpointsCellPercentDeviation=Module27.ResistanceTemperatureBreakpointsCellPercentDeviation  R0ThermalCell=Module27.R0ThermalCell Ohm  R0ThermalCellPercentDeviation=Module27.R0ThermalCellPercentDeviation  R1ThermalCell=Module27.R1ThermalCell Ohm  R1ThermalCellPercentDeviation=Module27.R1ThermalCellPercentDeviation  Tau1ThermalCell=Module27.Tau1ThermalCell s  Tau1ThermalCellPercentDeviation=Module27.Tau1ThermalCellPercentDeviation  BatteryThermalMassCell=Module27.BatteryThermalMassCell J/K  BatteryThermalMassCellPercentDeviation=Module27.BatteryThermalMassCellPercentDeviation  AmbientResistance=Module27.AmbientResistance K/W  P=2  S=6  socCell_specify=on  socCell_priority=High  socCell=Module27.socCell  socCell_nominal_specify=off  socCell_nominal_value=1  socCell_nominal_unit=1  batteryVoltage_specify=on  batteryVoltage_priority=None  batteryVoltage=Module27.batteryVoltage V  batteryVoltage_nominal_specify=off  batteryVoltage_nominal_value=1  batteryVoltage_nominal_unit=V  batteryCurrent_specify=on  batteryCurrent_priority=None  batteryCurrent=Module27.batteryCurrent A  batteryCurrent_nominal_specify=off  batteryCurrent_nominal_value=1  batteryCurrent_nominal_unit=A  numCycles_specify=on  numCycles_priority=High  numCycles=Module27.numCycles  numCycles_nominal_specify=off  numCycles_nominal_value=1  numCycles_nominal_unit=1  batteryTemperature_specify=on  batteryTemperature_priority=High  batteryTemperature=Module27.batteryTemperature K  batteryTemperature_nominal_specify=off  batteryTemperature_nominal_value=1  batteryTemperature_nominal_unit=K  vParallelAssembly_specify=on  vParallelAssembly_priority=None  vParallelAssembly=Module27.vParallelAssembly V  vParallelAssembly_nominal_specify=off  vParallelAssembly_nominal_value=1  vParallelAssembly_nominal_unit=V  socParallelAssembly_specify=on  socParallelAssembly_priority=None  socParallelAssembly=Module27.socParallelAssembly  socParallelAssembly_nominal_specify=off  socParallelAssembly_nominal_value=1  socParallelAssembly_nominal_unit=1
      settings: InternalSimscapePortConfiguration="{\"Bottom\":[{\"id\":\"n\",\"label\":\"-\",\"type\":\"foundation.electrical.electrical\"}],\"Left\":[{\"id\":\"AmbH\",\"label\":\"AmbH\",\"type\":\"foundation.thermal.thermal\"}],\"Right\":[],\"Top\":[{\"id\":\"p\",\"label\":\"+\",\"type\":\"foundation.electrical.electrical\"}]}"
  Module28 : thermalCoupledCellResolution_lib/Modules/ModuleType1  BatteryCapacityCell=Module28.BatteryCapacityCell A*hr  BatteryCapacityCellPercentDeviation=Module28.BatteryCapacityCellPercentDeviation  ExtrapolationMethodCell=simscape.enum.extrapolation.nearest  SOCBreakpointsCell=Module28.SOCBreakpointsCell  SOCBreakpointsCellPercentDeviation=Module28.SOCBreakpointsCellPercentDeviation  TemperatureBreakpointsCell=Module28.TemperatureBreakpointsCell K  TemperatureBreakpointsCellPercentDeviation=Module28.TemperatureBreakpointsCellPercentDeviation  OpenCircuitVoltageThermalCell=Module28.OpenCircuitVoltageThermalCell V  OpenCircuitVoltageThermalCellPercentDeviation=Module28.OpenCircuitVoltageThermalCellPercentDeviation  VoltageRangeCell=Module28.VoltageRangeCell V  VoltageRangeCellPercentDeviation=Module28.VoltageRangeCellPercentDeviation  ResistanceSOCBreakpointsCell=Module28.ResistanceSOCBreakpointsCell  ResistanceSOCBreakpointsCellPercentDeviation=Module28.ResistanceSOCBreakpointsCellPercentDeviation  ResistanceTemperatureBreakpointsCell=Module28.ResistanceTemperatureBreakpointsCell K  ResistanceTemperatureBreakpointsCellPercentDeviation=Module28.ResistanceTemperatureBreakpointsCellPercentDeviation  R0ThermalCell=Module28.R0ThermalCell Ohm  R0ThermalCellPercentDeviation=Module28.R0ThermalCellPercentDeviation  R1ThermalCell=Module28.R1ThermalCell Ohm  R1ThermalCellPercentDeviation=Module28.R1ThermalCellPercentDeviation  Tau1ThermalCell=Module28.Tau1ThermalCell s  Tau1ThermalCellPercentDeviation=Module28.Tau1ThermalCellPercentDeviation  BatteryThermalMassCell=Module28.BatteryThermalMassCell J/K  BatteryThermalMassCellPercentDeviation=Module28.BatteryThermalMassCellPercentDeviation  AmbientResistance=Module28.AmbientResistance K/W  P=2  S=6  socCell_specify=on  socCell_priority=High  socCell=Module28.socCell  socCell_nominal_specify=off  socCell_nominal_value=1  socCell_nominal_unit=1  batteryVoltage_specify=on  batteryVoltage_priority=None  batteryVoltage=Module28.batteryVoltage V  batteryVoltage_nominal_specify=off  batteryVoltage_nominal_value=1  batteryVoltage_nominal_unit=V  batteryCurrent_specify=on  batteryCurrent_priority=None  batteryCurrent=Module28.batteryCurrent A  batteryCurrent_nominal_specify=off  batteryCurrent_nominal_value=1  batteryCurrent_nominal_unit=A  numCycles_specify=on  numCycles_priority=High  numCycles=Module28.numCycles  numCycles_nominal_specify=off  numCycles_nominal_value=1  numCycles_nominal_unit=1  batteryTemperature_specify=on  batteryTemperature_priority=High  batteryTemperature=Module28.batteryTemperature K  batteryTemperature_nominal_specify=off  batteryTemperature_nominal_value=1  batteryTemperature_nominal_unit=K  vParallelAssembly_specify=on  vParallelAssembly_priority=None  vParallelAssembly=Module28.vParallelAssembly V  vParallelAssembly_nominal_specify=off  vParallelAssembly_nominal_value=1  vParallelAssembly_nominal_unit=V  socParallelAssembly_specify=on  socParallelAssembly_priority=None  socParallelAssembly=Module28.socParallelAssembly  socParallelAssembly_nominal_specify=off  socParallelAssembly_nominal_value=1  socParallelAssembly_nominal_unit=1
      settings: InternalSimscapePortConfiguration="{\"Bottom\":[{\"id\":\"n\",\"label\":\"-\",\"type\":\"foundation.electrical.electrical\"}],\"Left\":[{\"id\":\"AmbH\",\"label\":\"AmbH\",\"type\":\"foundation.thermal.thermal\"}],\"Right\":[],\"Top\":[{\"id\":\"p\",\"label\":\"+\",\"type\":\"foundation.electrical.electrical\"}]}"
  Module29 : thermalCoupledCellResolution_lib/Modules/ModuleType1  BatteryCapacityCell=Module29.BatteryCapacityCell A*hr  BatteryCapacityCellPercentDeviation=Module29.BatteryCapacityCellPercentDeviation  ExtrapolationMethodCell=simscape.enum.extrapolation.nearest  SOCBreakpointsCell=Module29.SOCBreakpointsCell  SOCBreakpointsCellPercentDeviation=Module29.SOCBreakpointsCellPercentDeviation  TemperatureBreakpointsCell=Module29.TemperatureBreakpointsCell K  TemperatureBreakpointsCellPercentDeviation=Module29.TemperatureBreakpointsCellPercentDeviation  OpenCircuitVoltageThermalCell=Module29.OpenCircuitVoltageThermalCell V  OpenCircuitVoltageThermalCellPercentDeviation=Module29.OpenCircuitVoltageThermalCellPercentDeviation  VoltageRangeCell=Module29.VoltageRangeCell V  VoltageRangeCellPercentDeviation=Module29.VoltageRangeCellPercentDeviation  ResistanceSOCBreakpointsCell=Module29.ResistanceSOCBreakpointsCell  ResistanceSOCBreakpointsCellPercentDeviation=Module29.ResistanceSOCBreakpointsCellPercentDeviation  ResistanceTemperatureBreakpointsCell=Module29.ResistanceTemperatureBreakpointsCell K  ResistanceTemperatureBreakpointsCellPercentDeviation=Module29.ResistanceTemperatureBreakpointsCellPercentDeviation  R0ThermalCell=Module29.R0ThermalCell Ohm  R0ThermalCellPercentDeviation=Module29.R0ThermalCellPercentDeviation  R1ThermalCell=Module29.R1ThermalCell Ohm  R1ThermalCellPercentDeviation=Module29.R1ThermalCellPercentDeviation  Tau1ThermalCell=Module29.Tau1ThermalCell s  Tau1ThermalCellPercentDeviation=Module29.Tau1ThermalCellPercentDeviation  BatteryThermalMassCell=Module29.BatteryThermalMassCell J/K  BatteryThermalMassCellPercentDeviation=Module29.BatteryThermalMassCellPercentDeviation  AmbientResistance=Module29.AmbientResistance K/W  P=2  S=6  socCell_specify=on  socCell_priority=High  socCell=Module29.socCell  socCell_nominal_specify=off  socCell_nominal_value=1  socCell_nominal_unit=1  batteryVoltage_specify=on  batteryVoltage_priority=None  batteryVoltage=Module29.batteryVoltage V  batteryVoltage_nominal_specify=off  batteryVoltage_nominal_value=1  batteryVoltage_nominal_unit=V  batteryCurrent_specify=on  batteryCurrent_priority=None  batteryCurrent=Module29.batteryCurrent A  batteryCurrent_nominal_specify=off  batteryCurrent_nominal_value=1  batteryCurrent_nominal_unit=A  numCycles_specify=on  numCycles_priority=High  numCycles=Module29.numCycles  numCycles_nominal_specify=off  numCycles_nominal_value=1  numCycles_nominal_unit=1  batteryTemperature_specify=on  batteryTemperature_priority=High  batteryTemperature=Module29.batteryTemperature K  batteryTemperature_nominal_specify=off  batteryTemperature_nominal_value=1  batteryTemperature_nominal_unit=K  vParallelAssembly_specify=on  vParallelAssembly_priority=None  vParallelAssembly=Module29.vParallelAssembly V  vParallelAssembly_nominal_specify=off  vParallelAssembly_nominal_value=1  vParallelAssembly_nominal_unit=V  socParallelAssembly_specify=on  socParallelAssembly_priority=None  socParallelAssembly=Module29.socParallelAssembly  socParallelAssembly_nominal_specify=off  socParallelAssembly_nominal_value=1  socParallelAssembly_nominal_unit=1
      settings: InternalSimscapePortConfiguration="{\"Bottom\":[{\"id\":\"n\",\"label\":\"-\",\"type\":\"foundation.electrical.electrical\"}],\"Left\":[{\"id\":\"AmbH\",\"label\":\"AmbH\",\"type\":\"foundation.thermal.thermal\"}],\"Right\":[],\"Top\":[{\"id\":\"p\",\"label\":\"+\",\"type\":\"foundation.electrical.electrical\"}]}"
  Module3 : thermalCoupledCellResolution_lib/Modules/ModuleType1  BatteryCapacityCell=Module03.BatteryCapacityCell A*hr  BatteryCapacityCellPercentDeviation=Module03.BatteryCapacityCellPercentDeviation  ExtrapolationMethodCell=simscape.enum.extrapolation.nearest  SOCBreakpointsCell=Module03.SOCBreakpointsCell  SOCBreakpointsCellPercentDeviation=Module03.SOCBreakpointsCellPercentDeviation  TemperatureBreakpointsCell=Module03.TemperatureBreakpointsCell K  TemperatureBreakpointsCellPercentDeviation=Module03.TemperatureBreakpointsCellPercentDeviation  OpenCircuitVoltageThermalCell=Module03.OpenCircuitVoltageThermalCell V  OpenCircuitVoltageThermalCellPercentDeviation=Module03.OpenCircuitVoltageThermalCellPercentDeviation  VoltageRangeCell=Module03.VoltageRangeCell V  VoltageRangeCellPercentDeviation=Module03.VoltageRangeCellPercentDeviation  ResistanceSOCBreakpointsCell=Module03.ResistanceSOCBreakpointsCell  ResistanceSOCBreakpointsCellPercentDeviation=Module03.ResistanceSOCBreakpointsCellPercentDeviation  ResistanceTemperatureBreakpointsCell=Module03.ResistanceTemperatureBreakpointsCell K  ResistanceTemperatureBreakpointsCellPercentDeviation=Module03.ResistanceTemperatureBreakpointsCellPercentDeviation  R0ThermalCell=Module03.R0ThermalCell Ohm  R0ThermalCellPercentDeviation=Module03.R0ThermalCellPercentDeviation  R1ThermalCell=Module03.R1ThermalCell Ohm  R1ThermalCellPercentDeviation=Module03.R1ThermalCellPercentDeviation  Tau1ThermalCell=Module03.Tau1ThermalCell s  Tau1ThermalCellPercentDeviation=Module03.Tau1ThermalCellPercentDeviation  BatteryThermalMassCell=Module03.BatteryThermalMassCell J/K  BatteryThermalMassCellPercentDeviation=Module03.BatteryThermalMassCellPercentDeviation  AmbientResistance=Module03.AmbientResistance K/W  P=2  S=6  socCell_specify=on  socCell_priority=High  socCell=Module03.socCell  socCell_nominal_specify=off  socCell_nominal_value=1  socCell_nominal_unit=1  batteryVoltage_specify=on  batteryVoltage_priority=None  batteryVoltage=Module03.batteryVoltage V  batteryVoltage_nominal_specify=off  batteryVoltage_nominal_value=1  batteryVoltage_nominal_unit=V  batteryCurrent_specify=on  batteryCurrent_priority=None  batteryCurrent=Module03.batteryCurrent A  batteryCurrent_nominal_specify=off  batteryCurrent_nominal_value=1  batteryCurrent_nominal_unit=A  numCycles_specify=on  numCycles_priority=High  numCycles=Module03.numCycles  numCycles_nominal_specify=off  numCycles_nominal_value=1  numCycles_nominal_unit=1  batteryTemperature_specify=on  batteryTemperature_priority=High  batteryTemperature=Module03.batteryTemperature K  batteryTemperature_nominal_specify=off  batteryTemperature_nominal_value=1  batteryTemperature_nominal_unit=K  vParallelAssembly_specify=on  vParallelAssembly_priority=None  vParallelAssembly=Module03.vParallelAssembly V  vParallelAssembly_nominal_specify=off  vParallelAssembly_nominal_value=1  vParallelAssembly_nominal_unit=V  socParallelAssembly_specify=on  socParallelAssembly_priority=None  socParallelAssembly=Module03.socParallelAssembly  socParallelAssembly_nominal_specify=off  socParallelAssembly_nominal_value=1  socParallelAssembly_nominal_unit=1
      settings: InternalSimscapePortConfiguration="{\"Bottom\":[{\"id\":\"n\",\"label\":\"-\",\"type\":\"foundation.electrical.electrical\"}],\"Left\":[{\"id\":\"AmbH\",\"label\":\"AmbH\",\"type\":\"foundation.thermal.thermal\"}],\"Right\":[],\"Top\":[{\"id\":\"p\",\"label\":\"+\",\"type\":\"foundation.electrical.electrical\"}]}"
  Module30 : thermalCoupledCellResolution_lib/Modules/ModuleType1  BatteryCapacityCell=Module30.BatteryCapacityCell A*hr  BatteryCapacityCellPercentDeviation=Module30.BatteryCapacityCellPercentDeviation  ExtrapolationMethodCell=simscape.enum.extrapolation.nearest  SOCBreakpointsCell=Module30.SOCBreakpointsCell  SOCBreakpointsCellPercentDeviation=Module30.SOCBreakpointsCellPercentDeviation  TemperatureBreakpointsCell=Module30.TemperatureBreakpointsCell K  TemperatureBreakpointsCellPercentDeviation=Module30.TemperatureBreakpointsCellPercentDeviation  OpenCircuitVoltageThermalCell=Module30.OpenCircuitVoltageThermalCell V  OpenCircuitVoltageThermalCellPercentDeviation=Module30.OpenCircuitVoltageThermalCellPercentDeviation  VoltageRangeCell=Module30.VoltageRangeCell V  VoltageRangeCellPercentDeviation=Module30.VoltageRangeCellPercentDeviation  ResistanceSOCBreakpointsCell=Module30.ResistanceSOCBreakpointsCell  ResistanceSOCBreakpointsCellPercentDeviation=Module30.ResistanceSOCBreakpointsCellPercentDeviation  ResistanceTemperatureBreakpointsCell=Module30.ResistanceTemperatureBreakpointsCell K  ResistanceTemperatureBreakpointsCellPercentDeviation=Module30.ResistanceTemperatureBreakpointsCellPercentDeviation  R0ThermalCell=Module30.R0ThermalCell Ohm  R0ThermalCellPercentDeviation=Module30.R0ThermalCellPercentDeviation  R1ThermalCell=Module30.R1ThermalCell Ohm  R1ThermalCellPercentDeviation=Module30.R1ThermalCellPercentDeviation  Tau1ThermalCell=Module30.Tau1ThermalCell s  Tau1ThermalCellPercentDeviation=Module30.Tau1ThermalCellPercentDeviation  BatteryThermalMassCell=Module30.BatteryThermalMassCell J/K  BatteryThermalMassCellPercentDeviation=Module30.BatteryThermalMassCellPercentDeviation  AmbientResistance=Module30.AmbientResistance K/W  P=2  S=6  socCell_specify=on  socCell_priority=High  socCell=Module30.socCell  socCell_nominal_specify=off  socCell_nominal_value=1  socCell_nominal_unit=1  batteryVoltage_specify=on  batteryVoltage_priority=None  batteryVoltage=Module30.batteryVoltage V  batteryVoltage_nominal_specify=off  batteryVoltage_nominal_value=1  batteryVoltage_nominal_unit=V  batteryCurrent_specify=on  batteryCurrent_priority=None  batteryCurrent=Module30.batteryCurrent A  batteryCurrent_nominal_specify=off  batteryCurrent_nominal_value=1  batteryCurrent_nominal_unit=A  numCycles_specify=on  numCycles_priority=High  numCycles=Module30.numCycles  numCycles_nominal_specify=off  numCycles_nominal_value=1  numCycles_nominal_unit=1  batteryTemperature_specify=on  batteryTemperature_priority=High  batteryTemperature=Module30.batteryTemperature K  batteryTemperature_nominal_specify=off  batteryTemperature_nominal_value=1  batteryTemperature_nominal_unit=K  vParallelAssembly_specify=on  vParallelAssembly_priority=None  vParallelAssembly=Module30.vParallelAssembly V  vParallelAssembly_nominal_specify=off  vParallelAssembly_nominal_value=1  vParallelAssembly_nominal_unit=V  socParallelAssembly_specify=on  socParallelAssembly_priority=None  socParallelAssembly=Module30.socParallelAssembly  socParallelAssembly_nominal_specify=off  socParallelAssembly_nominal_value=1  socParallelAssembly_nominal_unit=1
      settings: InternalSimscapePortConfiguration="{\"Bottom\":[{\"id\":\"n\",\"label\":\"-\",\"type\":\"foundation.electrical.electrical\"}],\"Left\":[{\"id\":\"AmbH\",\"label\":\"AmbH\",\"type\":\"foundation.thermal.thermal\"}],\"Right\":[],\"Top\":[{\"id\":\"p\",\"label\":\"+\",\"type\":\"foundation.electrical.electrical\"}]}"
  Module31 : thermalCoupledCellResolution_lib/Modules/ModuleType1  BatteryCapacityCell=Module31.BatteryCapacityCell A*hr  BatteryCapacityCellPercentDeviation=Module31.BatteryCapacityCellPercentDeviation  ExtrapolationMethodCell=simscape.enum.extrapolation.nearest  SOCBreakpointsCell=Module31.SOCBreakpointsCell  SOCBreakpointsCellPercentDeviation=Module31.SOCBreakpointsCellPercentDeviation  TemperatureBreakpointsCell=Module31.TemperatureBreakpointsCell K  TemperatureBreakpointsCellPercentDeviation=Module31.TemperatureBreakpointsCellPercentDeviation  OpenCircuitVoltageThermalCell=Module31.OpenCircuitVoltageThermalCell V  OpenCircuitVoltageThermalCellPercentDeviation=Module31.OpenCircuitVoltageThermalCellPercentDeviation  VoltageRangeCell=Module31.VoltageRangeCell V  VoltageRangeCellPercentDeviation=Module31.VoltageRangeCellPercentDeviation  ResistanceSOCBreakpointsCell=Module31.ResistanceSOCBreakpointsCell  ResistanceSOCBreakpointsCellPercentDeviation=Module31.ResistanceSOCBreakpointsCellPercentDeviation  ResistanceTemperatureBreakpointsCell=Module31.ResistanceTemperatureBreakpointsCell K  ResistanceTemperatureBreakpointsCellPercentDeviation=Module31.ResistanceTemperatureBreakpointsCellPercentDeviation  R0ThermalCell=Module31.R0ThermalCell Ohm  R0ThermalCellPercentDeviation=Module31.R0ThermalCellPercentDeviation  R1ThermalCell=Module31.R1ThermalCell Ohm  R1ThermalCellPercentDeviation=Module31.R1ThermalCellPercentDeviation  Tau1ThermalCell=Module31.Tau1ThermalCell s  Tau1ThermalCellPercentDeviation=Module31.Tau1ThermalCellPercentDeviation  BatteryThermalMassCell=Module31.BatteryThermalMassCell J/K  BatteryThermalMassCellPercentDeviation=Module31.BatteryThermalMassCellPercentDeviation  AmbientResistance=Module31.AmbientResistance K/W  P=2  S=6  socCell_specify=on  socCell_priority=High  socCell=Module31.socCell  socCell_nominal_specify=off  socCell_nominal_value=1  socCell_nominal_unit=1  batteryVoltage_specify=on  batteryVoltage_priority=None  batteryVoltage=Module31.batteryVoltage V  batteryVoltage_nominal_specify=off  batteryVoltage_nominal_value=1  batteryVoltage_nominal_unit=V  batteryCurrent_specify=on  batteryCurrent_priority=None  batteryCurrent=Module31.batteryCurrent A  batteryCurrent_nominal_specify=off  batteryCurrent_nominal_value=1  batteryCurrent_nominal_unit=A  numCycles_specify=on  numCycles_priority=High  numCycles=Module31.numCycles  numCycles_nominal_specify=off  numCycles_nominal_value=1  numCycles_nominal_unit=1  batteryTemperature_specify=on  batteryTemperature_priority=High  batteryTemperature=Module31.batteryTemperature K  batteryTemperature_nominal_specify=off  batteryTemperature_nominal_value=1  batteryTemperature_nominal_unit=K  vParallelAssembly_specify=on  vParallelAssembly_priority=None  vParallelAssembly=Module31.vParallelAssembly V  vParallelAssembly_nominal_specify=off  vParallelAssembly_nominal_value=1  vParallelAssembly_nominal_unit=V  socParallelAssembly_specify=on  socParallelAssembly_priority=None  socParallelAssembly=Module31.socParallelAssembly  socParallelAssembly_nominal_specify=off  socParallelAssembly_nominal_value=1  socParallelAssembly_nominal_unit=1
      settings: InternalSimscapePortConfiguration="{\"Bottom\":[{\"id\":\"n\",\"label\":\"-\",\"type\":\"foundation.electrical.electrical\"}],\"Left\":[{\"id\":\"AmbH\",\"label\":\"AmbH\",\"type\":\"foundation.thermal.thermal\"}],\"Right\":[],\"Top\":[{\"id\":\"p\",\"label\":\"+\",\"type\":\"foundation.electrical.electrical\"}]}"
  Module32 : thermalCoupledCellResolution_lib/Modules/ModuleType1  BatteryCapacityCell=Module32.BatteryCapacityCell A*hr  BatteryCapacityCellPercentDeviation=Module32.BatteryCapacityCellPercentDeviation  ExtrapolationMethodCell=simscape.enum.extrapolation.nearest  SOCBreakpointsCell=Module32.SOCBreakpointsCell  SOCBreakpointsCellPercentDeviation=Module32.SOCBreakpointsCellPercentDeviation  TemperatureBreakpointsCell=Module32.TemperatureBreakpointsCell K  TemperatureBreakpointsCellPercentDeviation=Module32.TemperatureBreakpointsCellPercentDeviation  OpenCircuitVoltageThermalCell=Module32.OpenCircuitVoltageThermalCell V  OpenCircuitVoltageThermalCellPercentDeviation=Module32.OpenCircuitVoltageThermalCellPercentDeviation  VoltageRangeCell=Module32.VoltageRangeCell V  VoltageRangeCellPercentDeviation=Module32.VoltageRangeCellPercentDeviation  ResistanceSOCBreakpointsCell=Module32.ResistanceSOCBreakpointsCell  ResistanceSOCBreakpointsCellPercentDeviation=Module32.ResistanceSOCBreakpointsCellPercentDeviation  ResistanceTemperatureBreakpointsCell=Module32.ResistanceTemperatureBreakpointsCell K  ResistanceTemperatureBreakpointsCellPercentDeviation=Module32.ResistanceTemperatureBreakpointsCellPercentDeviation  R0ThermalCell=Module32.R0ThermalCell Ohm  R0ThermalCellPercentDeviation=Module32.R0ThermalCellPercentDeviation  R1ThermalCell=Module32.R1ThermalCell Ohm  R1ThermalCellPercentDeviation=Module32.R1ThermalCellPercentDeviation  Tau1ThermalCell=Module32.Tau1ThermalCell s  Tau1ThermalCellPercentDeviation=Module32.Tau1ThermalCellPercentDeviation  BatteryThermalMassCell=Module32.BatteryThermalMassCell J/K  BatteryThermalMassCellPercentDeviation=Module32.BatteryThermalMassCellPercentDeviation  AmbientResistance=Module32.AmbientResistance K/W  P=2  S=6  socCell_specify=on  socCell_priority=High  socCell=Module32.socCell  socCell_nominal_specify=off  socCell_nominal_value=1  socCell_nominal_unit=1  batteryVoltage_specify=on  batteryVoltage_priority=None  batteryVoltage=Module32.batteryVoltage V  batteryVoltage_nominal_specify=off  batteryVoltage_nominal_value=1  batteryVoltage_nominal_unit=V  batteryCurrent_specify=on  batteryCurrent_priority=None  batteryCurrent=Module32.batteryCurrent A  batteryCurrent_nominal_specify=off  batteryCurrent_nominal_value=1  batteryCurrent_nominal_unit=A  numCycles_specify=on  numCycles_priority=High  numCycles=Module32.numCycles  numCycles_nominal_specify=off  numCycles_nominal_value=1  numCycles_nominal_unit=1  batteryTemperature_specify=on  batteryTemperature_priority=High  batteryTemperature=Module32.batteryTemperature K  batteryTemperature_nominal_specify=off  batteryTemperature_nominal_value=1  batteryTemperature_nominal_unit=K  vParallelAssembly_specify=on  vParallelAssembly_priority=None  vParallelAssembly=Module32.vParallelAssembly V  vParallelAssembly_nominal_specify=off  vParallelAssembly_nominal_value=1  vParallelAssembly_nominal_unit=V  socParallelAssembly_specify=on  socParallelAssembly_priority=None  socParallelAssembly=Module32.socParallelAssembly  socParallelAssembly_nominal_specify=off  socParallelAssembly_nominal_value=1  socParallelAssembly_nominal_unit=1
      settings: InternalSimscapePortConfiguration="{\"Bottom\":[{\"id\":\"n\",\"label\":\"-\",\"type\":\"foundation.electrical.electrical\"}],\"Left\":[{\"id\":\"AmbH\",\"label\":\"AmbH\",\"type\":\"foundation.thermal.thermal\"}],\"Right\":[],\"Top\":[{\"id\":\"p\",\"label\":\"+\",\"type\":\"foundation.electrical.electrical\"}]}"
  Module4 : thermalCoupledCellResolution_lib/Modules/ModuleType1  BatteryCapacityCell=Module04.BatteryCapacityCell A*hr  BatteryCapacityCellPercentDeviation=Module04.BatteryCapacityCellPercentDeviation  ExtrapolationMethodCell=simscape.enum.extrapolation.nearest  SOCBreakpointsCell=Module04.SOCBreakpointsCell  SOCBreakpointsCellPercentDeviation=Module04.SOCBreakpointsCellPercentDeviation  TemperatureBreakpointsCell=Module04.TemperatureBreakpointsCell K  TemperatureBreakpointsCellPercentDeviation=Module04.TemperatureBreakpointsCellPercentDeviation  OpenCircuitVoltageThermalCell=Module04.OpenCircuitVoltageThermalCell V  OpenCircuitVoltageThermalCellPercentDeviation=Module04.OpenCircuitVoltageThermalCellPercentDeviation  VoltageRangeCell=Module04.VoltageRangeCell V  VoltageRangeCellPercentDeviation=Module04.VoltageRangeCellPercentDeviation  ResistanceSOCBreakpointsCell=Module04.ResistanceSOCBreakpointsCell  ResistanceSOCBreakpointsCellPercentDeviation=Module04.ResistanceSOCBreakpointsCellPercentDeviation  ResistanceTemperatureBreakpointsCell=Module04.ResistanceTemperatureBreakpointsCell K  ResistanceTemperatureBreakpointsCellPercentDeviation=Module04.ResistanceTemperatureBreakpointsCellPercentDeviation  R0ThermalCell=Module04.R0ThermalCell Ohm  R0ThermalCellPercentDeviation=Module04.R0ThermalCellPercentDeviation  R1ThermalCell=Module04.R1ThermalCell Ohm  R1ThermalCellPercentDeviation=Module04.R1ThermalCellPercentDeviation  Tau1ThermalCell=Module04.Tau1ThermalCell s  Tau1ThermalCellPercentDeviation=Module04.Tau1ThermalCellPercentDeviation  BatteryThermalMassCell=Module04.BatteryThermalMassCell J/K  BatteryThermalMassCellPercentDeviation=Module04.BatteryThermalMassCellPercentDeviation  AmbientResistance=Module04.AmbientResistance K/W  P=2  S=6  socCell_specify=on  socCell_priority=High  socCell=Module04.socCell  socCell_nominal_specify=off  socCell_nominal_value=1  socCell_nominal_unit=1  batteryVoltage_specify=on  batteryVoltage_priority=None  batteryVoltage=Module04.batteryVoltage V  batteryVoltage_nominal_specify=off  batteryVoltage_nominal_value=1  batteryVoltage_nominal_unit=V  batteryCurrent_specify=on  batteryCurrent_priority=None  batteryCurrent=Module04.batteryCurrent A  batteryCurrent_nominal_specify=off  batteryCurrent_nominal_value=1  batteryCurrent_nominal_unit=A  numCycles_specify=on  numCycles_priority=High  numCycles=Module04.numCycles  numCycles_nominal_specify=off  numCycles_nominal_value=1  numCycles_nominal_unit=1  batteryTemperature_specify=on  batteryTemperature_priority=High  batteryTemperature=Module04.batteryTemperature K  batteryTemperature_nominal_specify=off  batteryTemperature_nominal_value=1  batteryTemperature_nominal_unit=K  vParallelAssembly_specify=on  vParallelAssembly_priority=None  vParallelAssembly=Module04.vParallelAssembly V  vParallelAssembly_nominal_specify=off  vParallelAssembly_nominal_value=1  vParallelAssembly_nominal_unit=V  socParallelAssembly_specify=on  socParallelAssembly_priority=None  socParallelAssembly=Module04.socParallelAssembly  socParallelAssembly_nominal_specify=off  socParallelAssembly_nominal_value=1  socParallelAssembly_nominal_unit=1
      settings: InternalSimscapePortConfiguration="{\"Bottom\":[{\"id\":\"n\",\"label\":\"-\",\"type\":\"foundation.electrical.electrical\"}],\"Left\":[{\"id\":\"AmbH\",\"label\":\"AmbH\",\"type\":\"foundation.thermal.thermal\"}],\"Right\":[],\"Top\":[{\"id\":\"p\",\"label\":\"+\",\"type\":\"foundation.electrical.electrical\"}]}"
  Module5 : thermalCoupledCellResolution_lib/Modules/ModuleType1  BatteryCapacityCell=Module05.BatteryCapacityCell A*hr  BatteryCapacityCellPercentDeviation=Module05.BatteryCapacityCellPercentDeviation  ExtrapolationMethodCell=simscape.enum.extrapolation.nearest  SOCBreakpointsCell=Module05.SOCBreakpointsCell  SOCBreakpointsCellPercentDeviation=Module05.SOCBreakpointsCellPercentDeviation  TemperatureBreakpointsCell=Module05.TemperatureBreakpointsCell K  TemperatureBreakpointsCellPercentDeviation=Module05.TemperatureBreakpointsCellPercentDeviation  OpenCircuitVoltageThermalCell=Module05.OpenCircuitVoltageThermalCell V  OpenCircuitVoltageThermalCellPercentDeviation=Module05.OpenCircuitVoltageThermalCellPercentDeviation  VoltageRangeCell=Module05.VoltageRangeCell V  VoltageRangeCellPercentDeviation=Module05.VoltageRangeCellPercentDeviation  ResistanceSOCBreakpointsCell=Module05.ResistanceSOCBreakpointsCell  ResistanceSOCBreakpointsCellPercentDeviation=Module05.ResistanceSOCBreakpointsCellPercentDeviation  ResistanceTemperatureBreakpointsCell=Module05.ResistanceTemperatureBreakpointsCell K  ResistanceTemperatureBreakpointsCellPercentDeviation=Module05.ResistanceTemperatureBreakpointsCellPercentDeviation  R0ThermalCell=Module05.R0ThermalCell Ohm  R0ThermalCellPercentDeviation=Module05.R0ThermalCellPercentDeviation  R1ThermalCell=Module05.R1ThermalCell Ohm  R1ThermalCellPercentDeviation=Module05.R1ThermalCellPercentDeviation  Tau1ThermalCell=Module05.Tau1ThermalCell s  Tau1ThermalCellPercentDeviation=Module05.Tau1ThermalCellPercentDeviation  BatteryThermalMassCell=Module05.BatteryThermalMassCell J/K  BatteryThermalMassCellPercentDeviation=Module05.BatteryThermalMassCellPercentDeviation  AmbientResistance=Module05.AmbientResistance K/W  P=2  S=6  socCell_specify=on  socCell_priority=High  socCell=Module05.socCell  socCell_nominal_specify=off  socCell_nominal_value=1  socCell_nominal_unit=1  batteryVoltage_specify=on  batteryVoltage_priority=None  batteryVoltage=Module05.batteryVoltage V  batteryVoltage_nominal_specify=off  batteryVoltage_nominal_value=1  batteryVoltage_nominal_unit=V  batteryCurrent_specify=on  batteryCurrent_priority=None  batteryCurrent=Module05.batteryCurrent A  batteryCurrent_nominal_specify=off  batteryCurrent_nominal_value=1  batteryCurrent_nominal_unit=A  numCycles_specify=on  numCycles_priority=High  numCycles=Module05.numCycles  numCycles_nominal_specify=off  numCycles_nominal_value=1  numCycles_nominal_unit=1  batteryTemperature_specify=on  batteryTemperature_priority=High  batteryTemperature=Module05.batteryTemperature K  batteryTemperature_nominal_specify=off  batteryTemperature_nominal_value=1  batteryTemperature_nominal_unit=K  vParallelAssembly_specify=on  vParallelAssembly_priority=None  vParallelAssembly=Module05.vParallelAssembly V  vParallelAssembly_nominal_specify=off  vParallelAssembly_nominal_value=1  vParallelAssembly_nominal_unit=V  socParallelAssembly_specify=on  socParallelAssembly_priority=None  socParallelAssembly=Module05.socParallelAssembly  socParallelAssembly_nominal_specify=off  socParallelAssembly_nominal_value=1  socParallelAssembly_nominal_unit=1
      settings: InternalSimscapePortConfiguration="{\"Bottom\":[{\"id\":\"n\",\"label\":\"-\",\"type\":\"foundation.electrical.electrical\"}],\"Left\":[{\"id\":\"AmbH\",\"label\":\"AmbH\",\"type\":\"foundation.thermal.thermal\"}],\"Right\":[],\"Top\":[{\"id\":\"p\",\"label\":\"+\",\"type\":\"foundation.electrical.electrical\"}]}"
  Module6 : thermalCoupledCellResolution_lib/Modules/ModuleType1  BatteryCapacityCell=Module06.BatteryCapacityCell A*hr  BatteryCapacityCellPercentDeviation=Module06.BatteryCapacityCellPercentDeviation  ExtrapolationMethodCell=simscape.enum.extrapolation.nearest  SOCBreakpointsCell=Module06.SOCBreakpointsCell  SOCBreakpointsCellPercentDeviation=Module06.SOCBreakpointsCellPercentDeviation  TemperatureBreakpointsCell=Module06.TemperatureBreakpointsCell K  TemperatureBreakpointsCellPercentDeviation=Module06.TemperatureBreakpointsCellPercentDeviation  OpenCircuitVoltageThermalCell=Module06.OpenCircuitVoltageThermalCell V  OpenCircuitVoltageThermalCellPercentDeviation=Module06.OpenCircuitVoltageThermalCellPercentDeviation  VoltageRangeCell=Module06.VoltageRangeCell V  VoltageRangeCellPercentDeviation=Module06.VoltageRangeCellPercentDeviation  ResistanceSOCBreakpointsCell=Module06.ResistanceSOCBreakpointsCell  ResistanceSOCBreakpointsCellPercentDeviation=Module06.ResistanceSOCBreakpointsCellPercentDeviation  ResistanceTemperatureBreakpointsCell=Module06.ResistanceTemperatureBreakpointsCell K  ResistanceTemperatureBreakpointsCellPercentDeviation=Module06.ResistanceTemperatureBreakpointsCellPercentDeviation  R0ThermalCell=Module06.R0ThermalCell Ohm  R0ThermalCellPercentDeviation=Module06.R0ThermalCellPercentDeviation  R1ThermalCell=Module06.R1ThermalCell Ohm  R1ThermalCellPercentDeviation=Module06.R1ThermalCellPercentDeviation  Tau1ThermalCell=Module06.Tau1ThermalCell s  Tau1ThermalCellPercentDeviation=Module06.Tau1ThermalCellPercentDeviation  BatteryThermalMassCell=Module06.BatteryThermalMassCell J/K  BatteryThermalMassCellPercentDeviation=Module06.BatteryThermalMassCellPercentDeviation  AmbientResistance=Module06.AmbientResistance K/W  P=2  S=6  socCell_specify=on  socCell_priority=High  socCell=Module06.socCell  socCell_nominal_specify=off  socCell_nominal_value=1  socCell_nominal_unit=1  batteryVoltage_specify=on  batteryVoltage_priority=None  batteryVoltage=Module06.batteryVoltage V  batteryVoltage_nominal_specify=off  batteryVoltage_nominal_value=1  batteryVoltage_nominal_unit=V  batteryCurrent_specify=on  batteryCurrent_priority=None  batteryCurrent=Module06.batteryCurrent A  batteryCurrent_nominal_specify=off  batteryCurrent_nominal_value=1  batteryCurrent_nominal_unit=A  numCycles_specify=on  numCycles_priority=High  numCycles=Module06.numCycles  numCycles_nominal_specify=off  numCycles_nominal_value=1  numCycles_nominal_unit=1  batteryTemperature_specify=on  batteryTemperature_priority=High  batteryTemperature=Module06.batteryTemperature K  batteryTemperature_nominal_specify=off  batteryTemperature_nominal_value=1  batteryTemperature_nominal_unit=K  vParallelAssembly_specify=on  vParallelAssembly_priority=None  vParallelAssembly=Module06.vParallelAssembly V  vParallelAssembly_nominal_specify=off  vParallelAssembly_nominal_value=1  vParallelAssembly_nominal_unit=V  socParallelAssembly_specify=on  socParallelAssembly_priority=None  socParallelAssembly=Module06.socParallelAssembly  socParallelAssembly_nominal_specify=off  socParallelAssembly_nominal_value=1  socParallelAssembly_nominal_unit=1
      settings: InternalSimscapePortConfiguration="{\"Bottom\":[{\"id\":\"n\",\"label\":\"-\",\"type\":\"foundation.electrical.electrical\"}],\"Left\":[{\"id\":\"AmbH\",\"label\":\"AmbH\",\"type\":\"foundation.thermal.thermal\"}],\"Right\":[],\"Top\":[{\"id\":\"p\",\"label\":\"+\",\"type\":\"foundation.electrical.electrical\"}]}"
  Module7 : thermalCoupledCellResolution_lib/Modules/ModuleType1  BatteryCapacityCell=Module07.BatteryCapacityCell A*hr  BatteryCapacityCellPercentDeviation=Module07.BatteryCapacityCellPercentDeviation  ExtrapolationMethodCell=simscape.enum.extrapolation.nearest  SOCBreakpointsCell=Module07.SOCBreakpointsCell  SOCBreakpointsCellPercentDeviation=Module07.SOCBreakpointsCellPercentDeviation  TemperatureBreakpointsCell=Module07.TemperatureBreakpointsCell K  TemperatureBreakpointsCellPercentDeviation=Module07.TemperatureBreakpointsCellPercentDeviation  OpenCircuitVoltageThermalCell=Module07.OpenCircuitVoltageThermalCell V  OpenCircuitVoltageThermalCellPercentDeviation=Module07.OpenCircuitVoltageThermalCellPercentDeviation  VoltageRangeCell=Module07.VoltageRangeCell V  VoltageRangeCellPercentDeviation=Module07.VoltageRangeCellPercentDeviation  ResistanceSOCBreakpointsCell=Module07.ResistanceSOCBreakpointsCell  ResistanceSOCBreakpointsCellPercentDeviation=Module07.ResistanceSOCBreakpointsCellPercentDeviation  ResistanceTemperatureBreakpointsCell=Module07.ResistanceTemperatureBreakpointsCell K  ResistanceTemperatureBreakpointsCellPercentDeviation=Module07.ResistanceTemperatureBreakpointsCellPercentDeviation  R0ThermalCell=Module07.R0ThermalCell Ohm  R0ThermalCellPercentDeviation=Module07.R0ThermalCellPercentDeviation  R1ThermalCell=Module07.R1ThermalCell Ohm  R1ThermalCellPercentDeviation=Module07.R1ThermalCellPercentDeviation  Tau1ThermalCell=Module07.Tau1ThermalCell s  Tau1ThermalCellPercentDeviation=Module07.Tau1ThermalCellPercentDeviation  BatteryThermalMassCell=Module07.BatteryThermalMassCell J/K  BatteryThermalMassCellPercentDeviation=Module07.BatteryThermalMassCellPercentDeviation  AmbientResistance=Module07.AmbientResistance K/W  P=2  S=6  socCell_specify=on  socCell_priority=High  socCell=Module07.socCell  socCell_nominal_specify=off  socCell_nominal_value=1  socCell_nominal_unit=1  batteryVoltage_specify=on  batteryVoltage_priority=None  batteryVoltage=Module07.batteryVoltage V  batteryVoltage_nominal_specify=off  batteryVoltage_nominal_value=1  batteryVoltage_nominal_unit=V  batteryCurrent_specify=on  batteryCurrent_priority=None  batteryCurrent=Module07.batteryCurrent A  batteryCurrent_nominal_specify=off  batteryCurrent_nominal_value=1  batteryCurrent_nominal_unit=A  numCycles_specify=on  numCycles_priority=High  numCycles=Module07.numCycles  numCycles_nominal_specify=off  numCycles_nominal_value=1  numCycles_nominal_unit=1  batteryTemperature_specify=on  batteryTemperature_priority=High  batteryTemperature=Module07.batteryTemperature K  batteryTemperature_nominal_specify=off  batteryTemperature_nominal_value=1  batteryTemperature_nominal_unit=K  vParallelAssembly_specify=on  vParallelAssembly_priority=None  vParallelAssembly=Module07.vParallelAssembly V  vParallelAssembly_nominal_specify=off  vParallelAssembly_nominal_value=1  vParallelAssembly_nominal_unit=V  socParallelAssembly_specify=on  socParallelAssembly_priority=None  socParallelAssembly=Module07.socParallelAssembly  socParallelAssembly_nominal_specify=off  socParallelAssembly_nominal_value=1  socParallelAssembly_nominal_unit=1
      settings: InternalSimscapePortConfiguration="{\"Bottom\":[{\"id\":\"n\",\"label\":\"-\",\"type\":\"foundation.electrical.electrical\"}],\"Left\":[{\"id\":\"AmbH\",\"label\":\"AmbH\",\"type\":\"foundation.thermal.thermal\"}],\"Right\":[],\"Top\":[{\"id\":\"p\",\"label\":\"+\",\"type\":\"foundation.electrical.electrical\"}]}"
  Module8 : thermalCoupledCellResolution_lib/Modules/ModuleType1  BatteryCapacityCell=Module08.BatteryCapacityCell A*hr  BatteryCapacityCellPercentDeviation=Module08.BatteryCapacityCellPercentDeviation  ExtrapolationMethodCell=simscape.enum.extrapolation.nearest  SOCBreakpointsCell=Module08.SOCBreakpointsCell  SOCBreakpointsCellPercentDeviation=Module08.SOCBreakpointsCellPercentDeviation  TemperatureBreakpointsCell=Module08.TemperatureBreakpointsCell K  TemperatureBreakpointsCellPercentDeviation=Module08.TemperatureBreakpointsCellPercentDeviation  OpenCircuitVoltageThermalCell=Module08.OpenCircuitVoltageThermalCell V  OpenCircuitVoltageThermalCellPercentDeviation=Module08.OpenCircuitVoltageThermalCellPercentDeviation  VoltageRangeCell=Module08.VoltageRangeCell V  VoltageRangeCellPercentDeviation=Module08.VoltageRangeCellPercentDeviation  ResistanceSOCBreakpointsCell=Module08.ResistanceSOCBreakpointsCell  ResistanceSOCBreakpointsCellPercentDeviation=Module08.ResistanceSOCBreakpointsCellPercentDeviation  ResistanceTemperatureBreakpointsCell=Module08.ResistanceTemperatureBreakpointsCell K  ResistanceTemperatureBreakpointsCellPercentDeviation=Module08.ResistanceTemperatureBreakpointsCellPercentDeviation  R0ThermalCell=Module08.R0ThermalCell Ohm  R0ThermalCellPercentDeviation=Module08.R0ThermalCellPercentDeviation  R1ThermalCell=Module08.R1ThermalCell Ohm  R1ThermalCellPercentDeviation=Module08.R1ThermalCellPercentDeviation  Tau1ThermalCell=Module08.Tau1ThermalCell s  Tau1ThermalCellPercentDeviation=Module08.Tau1ThermalCellPercentDeviation  BatteryThermalMassCell=Module08.BatteryThermalMassCell J/K  BatteryThermalMassCellPercentDeviation=Module08.BatteryThermalMassCellPercentDeviation  AmbientResistance=Module08.AmbientResistance K/W  P=2  S=6  socCell_specify=on  socCell_priority=High  socCell=Module08.socCell  socCell_nominal_specify=off  socCell_nominal_value=1  socCell_nominal_unit=1  batteryVoltage_specify=on  batteryVoltage_priority=None  batteryVoltage=Module08.batteryVoltage V  batteryVoltage_nominal_specify=off  batteryVoltage_nominal_value=1  batteryVoltage_nominal_unit=V  batteryCurrent_specify=on  batteryCurrent_priority=None  batteryCurrent=Module08.batteryCurrent A  batteryCurrent_nominal_specify=off  batteryCurrent_nominal_value=1  batteryCurrent_nominal_unit=A  numCycles_specify=on  numCycles_priority=High  numCycles=Module08.numCycles  numCycles_nominal_specify=off  numCycles_nominal_value=1  numCycles_nominal_unit=1  batteryTemperature_specify=on  batteryTemperature_priority=High  batteryTemperature=Module08.batteryTemperature K  batteryTemperature_nominal_specify=off  batteryTemperature_nominal_value=1  batteryTemperature_nominal_unit=K  vParallelAssembly_specify=on  vParallelAssembly_priority=None  vParallelAssembly=Module08.vParallelAssembly V  vParallelAssembly_nominal_specify=off  vParallelAssembly_nominal_value=1  vParallelAssembly_nominal_unit=V  socParallelAssembly_specify=on  socParallelAssembly_priority=None  socParallelAssembly=Module08.socParallelAssembly  socParallelAssembly_nominal_specify=off  socParallelAssembly_nominal_value=1  socParallelAssembly_nominal_unit=1
      settings: InternalSimscapePortConfiguration="{\"Bottom\":[{\"id\":\"n\",\"label\":\"-\",\"type\":\"foundation.electrical.electrical\"}],\"Left\":[{\"id\":\"AmbH\",\"label\":\"AmbH\",\"type\":\"foundation.thermal.thermal\"}],\"Right\":[],\"Top\":[{\"id\":\"p\",\"label\":\"+\",\"type\":\"foundation.electrical.electrical\"}]}"
  Module9 : thermalCoupledCellResolution_lib/Modules/ModuleType1  BatteryCapacityCell=Module09.BatteryCapacityCell A*hr  BatteryCapacityCellPercentDeviation=Module09.BatteryCapacityCellPercentDeviation  ExtrapolationMethodCell=simscape.enum.extrapolation.nearest  SOCBreakpointsCell=Module09.SOCBreakpointsCell  SOCBreakpointsCellPercentDeviation=Module09.SOCBreakpointsCellPercentDeviation  TemperatureBreakpointsCell=Module09.TemperatureBreakpointsCell K  TemperatureBreakpointsCellPercentDeviation=Module09.TemperatureBreakpointsCellPercentDeviation  OpenCircuitVoltageThermalCell=Module09.OpenCircuitVoltageThermalCell V  OpenCircuitVoltageThermalCellPercentDeviation=Module09.OpenCircuitVoltageThermalCellPercentDeviation  VoltageRangeCell=Module09.VoltageRangeCell V  VoltageRangeCellPercentDeviation=Module09.VoltageRangeCellPercentDeviation  ResistanceSOCBreakpointsCell=Module09.ResistanceSOCBreakpointsCell  ResistanceSOCBreakpointsCellPercentDeviation=Module09.ResistanceSOCBreakpointsCellPercentDeviation  ResistanceTemperatureBreakpointsCell=Module09.ResistanceTemperatureBreakpointsCell K  ResistanceTemperatureBreakpointsCellPercentDeviation=Module09.ResistanceTemperatureBreakpointsCellPercentDeviation  R0ThermalCell=Module09.R0ThermalCell Ohm  R0ThermalCellPercentDeviation=Module09.R0ThermalCellPercentDeviation  R1ThermalCell=Module09.R1ThermalCell Ohm  R1ThermalCellPercentDeviation=Module09.R1ThermalCellPercentDeviation  Tau1ThermalCell=Module09.Tau1ThermalCell s  Tau1ThermalCellPercentDeviation=Module09.Tau1ThermalCellPercentDeviation  BatteryThermalMassCell=Module09.BatteryThermalMassCell J/K  BatteryThermalMassCellPercentDeviation=Module09.BatteryThermalMassCellPercentDeviation  AmbientResistance=Module09.AmbientResistance K/W  P=2  S=6  socCell_specify=on  socCell_priority=High  socCell=Module09.socCell  socCell_nominal_specify=off  socCell_nominal_value=1  socCell_nominal_unit=1  batteryVoltage_specify=on  batteryVoltage_priority=None  batteryVoltage=Module09.batteryVoltage V  batteryVoltage_nominal_specify=off  batteryVoltage_nominal_value=1  batteryVoltage_nominal_unit=V  batteryCurrent_specify=on  batteryCurrent_priority=None  batteryCurrent=Module09.batteryCurrent A  batteryCurrent_nominal_specify=off  batteryCurrent_nominal_value=1  batteryCurrent_nominal_unit=A  numCycles_specify=on  numCycles_priority=High  numCycles=Module09.numCycles  numCycles_nominal_specify=off  numCycles_nominal_value=1  numCycles_nominal_unit=1  batteryTemperature_specify=on  batteryTemperature_priority=High  batteryTemperature=Module09.batteryTemperature K  batteryTemperature_nominal_specify=off  batteryTemperature_nominal_value=1  batteryTemperature_nominal_unit=K  vParallelAssembly_specify=on  vParallelAssembly_priority=None  vParallelAssembly=Module09.vParallelAssembly V  vParallelAssembly_nominal_specify=off  vParallelAssembly_nominal_value=1  vParallelAssembly_nominal_unit=V  socParallelAssembly_specify=on  socParallelAssembly_priority=None  socParallelAssembly=Module09.socParallelAssembly  socParallelAssembly_nominal_specify=off  socParallelAssembly_nominal_value=1  socParallelAssembly_nominal_unit=1
      settings: InternalSimscapePortConfiguration="{\"Bottom\":[{\"id\":\"n\",\"label\":\"-\",\"type\":\"foundation.electrical.electrical\"}],\"Left\":[{\"id\":\"AmbH\",\"label\":\"AmbH\",\"type\":\"foundation.thermal.thermal\"}],\"Right\":[],\"Top\":[{\"id\":\"p\",\"label\":\"+\",\"type\":\"foundation.electrical.electrical\"}]}"
  MyProbeBlock1 : SimscapeProbe  BoundBlock=1  Variables="{\"batteryCurrent\":{\"Probing\":\"ON\"},\"batteryTemperature\":{\"Probing\":\"ON\"},\"batteryVoltage\":{\"Probing\":\"ON\"},\"socCell\":{\"Probing\":\"ON\"}}"
  MyProbeBlock10 : SimscapeProbe  BoundBlock=10  Variables="{\"batteryCurrent\":{\"Probing\":\"ON\"},\"batteryTemperature\":{\"Probing\":\"ON\"},\"batteryVoltage\":{\"Probing\":\"ON\"},\"socCell\":{\"Probing\":\"ON\"}}"
  MyProbeBlock11 : SimscapeProbe  BoundBlock=11  Variables="{\"batteryCurrent\":{\"Probing\":\"ON\"},\"batteryTemperature\":{\"Probing\":\"ON\"},\"batteryVoltage\":{\"Probing\":\"ON\"},\"socCell\":{\"Probing\":\"ON\"}}"
  MyProbeBlock12 : SimscapeProbe  BoundBlock=12  Variables="{\"batteryCurrent\":{\"Probing\":\"ON\"},\"batteryTemperature\":{\"Probing\":\"ON\"},\"batteryVoltage\":{\"Probing\":\"ON\"},\"socCell\":{\"Probing\":\"ON\"}}"
  MyProbeBlock13 : SimscapeProbe  BoundBlock=13  Variables="{\"batteryCurrent\":{\"Probing\":\"ON\"},\"batteryTemperature\":{\"Probing\":\"ON\"},\"batteryVoltage\":{\"Probing\":\"ON\"},\"socCell\":{\"Probing\":\"ON\"}}"
  MyProbeBlock14 : SimscapeProbe  BoundBlock=14  Variables="{\"batteryCurrent\":{\"Probing\":\"ON\"},\"batteryTemperature\":{\"Probing\":\"ON\"},\"batteryVoltage\":{\"Probing\":\"ON\"},\"socCell\":{\"Probing\":\"ON\"}}"
  MyProbeBlock15 : SimscapeProbe  BoundBlock=15  Variables="{\"batteryCurrent\":{\"Probing\":\"ON\"},\"batteryTemperature\":{\"Probing\":\"ON\"},\"batteryVoltage\":{\"Probing\":\"ON\"},\"socCell\":{\"Probing\":\"ON\"}}"
  MyProbeBlock16 : SimscapeProbe  BoundBlock=16  Variables="{\"batteryCurrent\":{\"Probing\":\"ON\"},\"batteryTemperature\":{\"Probing\":\"ON\"},\"batteryVoltage\":{\"Probing\":\"ON\"},\"socCell\":{\"Probing\":\"ON\"}}"
  MyProbeBlock17 : SimscapeProbe  BoundBlock=17  Variables="{\"batteryCurrent\":{\"Probing\":\"ON\"},\"batteryTemperature\":{\"Probing\":\"ON\"},\"batteryVoltage\":{\"Probing\":\"ON\"},\"socCell\":{\"Probing\":\"ON\"}}"
  MyProbeBlock18 : SimscapeProbe  BoundBlock=18  Variables="{\"batteryCurrent\":{\"Probing\":\"ON\"},\"batteryTemperature\":{\"Probing\":\"ON\"},\"batteryVoltage\":{\"Probing\":\"ON\"},\"socCell\":{\"Probing\":\"ON\"}}"
  MyProbeBlock19 : SimscapeProbe  BoundBlock=19  Variables="{\"batteryCurrent\":{\"Probing\":\"ON\"},\"batteryTemperature\":{\"Probing\":\"ON\"},\"batteryVoltage\":{\"Probing\":\"ON\"},\"socCell\":{\"Probing\":\"ON\"}}"
  MyProbeBlock2 : SimscapeProbe  BoundBlock=2  Variables="{\"batteryCurrent\":{\"Probing\":\"ON\"},\"batteryTemperature\":{\"Probing\":\"ON\"},\"batteryVoltage\":{\"Probing\":\"ON\"},\"socCell\":{\"Probing\":\"ON\"}}"
  MyProbeBlock20 : SimscapeProbe  BoundBlock=20  Variables="{\"batteryCurrent\":{\"Probing\":\"ON\"},\"batteryTemperature\":{\"Probing\":\"ON\"},\"batteryVoltage\":{\"Probing\":\"ON\"},\"socCell\":{\"Probing\":\"ON\"}}"
  MyProbeBlock21 : SimscapeProbe  BoundBlock=21  Variables="{\"batteryCurrent\":{\"Probing\":\"ON\"},\"batteryTemperature\":{\"Probing\":\"ON\"},\"batteryVoltage\":{\"Probing\":\"ON\"},\"socCell\":{\"Probing\":\"ON\"}}"
  MyProbeBlock22 : SimscapeProbe  BoundBlock=22  Variables="{\"batteryCurrent\":{\"Probing\":\"ON\"},\"batteryTemperature\":{\"Probing\":\"ON\"},\"batteryVoltage\":{\"Probing\":\"ON\"},\"socCell\":{\"Probing\":\"ON\"}}"
  MyProbeBlock23 : SimscapeProbe  BoundBlock=23  Variables="{\"batteryCurrent\":{\"Probing\":\"ON\"},\"batteryTemperature\":{\"Probing\":\"ON\"},\"batteryVoltage\":{\"Probing\":\"ON\"},\"socCell\":{\"Probing\":\"ON\"}}"
  MyProbeBlock24 : SimscapeProbe  BoundBlock=24  Variables="{\"batteryCurrent\":{\"Probing\":\"ON\"},\"batteryTemperature\":{\"Probing\":\"ON\"},\"batteryVoltage\":{\"Probing\":\"ON\"},\"socCell\":{\"Probing\":\"ON\"}}"
  MyProbeBlock25 : SimscapeProbe  BoundBlock=25  Variables="{\"batteryCurrent\":{\"Probing\":\"ON\"},\"batteryTemperature\":{\"Probing\":\"ON\"},\"batteryVoltage\":{\"Probing\":\"ON\"},\"socCell\":{\"Probing\":\"ON\"}}"
  MyProbeBlock26 : SimscapeProbe  BoundBlock=26  Variables="{\"batteryCurrent\":{\"Probing\":\"ON\"},\"batteryTemperature\":{\"Probing\":\"ON\"},\"batteryVoltage\":{\"Probing\":\"ON\"},\"socCell\":{\"Probing\":\"ON\"}}"
  MyProbeBlock27 : SimscapeProbe  BoundBlock=27  Variables="{\"batteryCurrent\":{\"Probing\":\"ON\"},\"batteryTemperature\":{\"Probing\":\"ON\"},\"batteryVoltage\":{\"Probing\":\"ON\"},\"socCell\":{\"Probing\":\"ON\"}}"
  MyProbeBlock28 : SimscapeProbe  BoundBlock=28  Variables="{\"batteryCurrent\":{\"Probing\":\"ON\"},\"batteryTemperature\":{\"Probing\":\"ON\"},\"batteryVoltage\":{\"Probing\":\"ON\"},\"socCell\":{\"Probing\":\"ON\"}}"
  MyProbeBlock29 : SimscapeProbe  BoundBlock=29  Variables="{\"batteryCurrent\":{\"Probing\":\"ON\"},\"batteryTemperature\":{\"Probing\":\"ON\"},\"batteryVoltage\":{\"Probing\":\"ON\"},\"socCell\":{\"Probing\":\"ON\"}}"
  MyProbeBlock3 : SimscapeProbe  BoundBlock=3  Variables="{\"batteryCurrent\":{\"Probing\":\"ON\"},\"batteryTemperature\":{\"Probing\":\"ON\"},\"batteryVoltage\":{\"Probing\":\"ON\"},\"socCell\":{\"Probing\":\"ON\"}}"
  MyProbeBlock30 : SimscapeProbe  BoundBlock=30  Variables="{\"batteryCurrent\":{\"Probing\":\"ON\"},\"batteryTemperature\":{\"Probing\":\"ON\"},\"batteryVoltage\":{\"Probing\":\"ON\"},\"socCell\":{\"Probing\":\"ON\"}}"
  MyProbeBlock31 : SimscapeProbe  BoundBlock=31  Variables="{\"batteryCurrent\":{\"Probing\":\"ON\"},\"batteryTemperature\":{\"Probing\":\"ON\"},\"batteryVoltage\":{\"Probing\":\"ON\"},\"socCell\":{\"Probing\":\"ON\"}}"
  MyProbeBlock32 : SimscapeProbe  BoundBlock=32  Variables="{\"batteryCurrent\":{\"Probing\":\"ON\"},\"batteryTemperature\":{\"Probing\":\"ON\"},\"batteryVoltage\":{\"Probing\":\"ON\"},\"socCell\":{\"Probing\":\"ON\"}}"
  MyProbeBlock4 : SimscapeProbe  BoundBlock=4  Variables="{\"batteryCurrent\":{\"Probing\":\"ON\"},\"batteryTemperature\":{\"Probing\":\"ON\"},\"batteryVoltage\":{\"Probing\":\"ON\"},\"socCell\":{\"Probing\":\"ON\"}}"
  MyProbeBlock5 : SimscapeProbe  BoundBlock=5  Variables="{\"batteryCurrent\":{\"Probing\":\"ON\"},\"batteryTemperature\":{\"Probing\":\"ON\"},\"batteryVoltage\":{\"Probing\":\"ON\"},\"socCell\":{\"Probing\":\"ON\"}}"
  MyProbeBlock6 : SimscapeProbe  BoundBlock=6  Variables="{\"batteryCurrent\":{\"Probing\":\"ON\"},\"batteryTemperature\":{\"Probing\":\"ON\"},\"batteryVoltage\":{\"Probing\":\"ON\"},\"socCell\":{\"Probing\":\"ON\"}}"
  MyProbeBlock7 : SimscapeProbe  BoundBlock=7  Variables="{\"batteryCurrent\":{\"Probing\":\"ON\"},\"batteryTemperature\":{\"Probing\":\"ON\"},\"batteryVoltage\":{\"Probing\":\"ON\"},\"socCell\":{\"Probing\":\"ON\"}}"
  MyProbeBlock8 : SimscapeProbe  BoundBlock=8  Variables="{\"batteryCurrent\":{\"Probing\":\"ON\"},\"batteryTemperature\":{\"Probing\":\"ON\"},\"batteryVoltage\":{\"Probing\":\"ON\"},\"socCell\":{\"Probing\":\"ON\"}}"
  MyProbeBlock9 : SimscapeProbe  BoundBlock=9  Variables="{\"batteryCurrent\":{\"Probing\":\"ON\"},\"batteryTemperature\":{\"Probing\":\"ON\"},\"batteryVoltage\":{\"Probing\":\"ON\"},\"socCell\":{\"Probing\":\"ON\"}}"
  PackProbe : SimscapeProbe  BoundBlock=98  Variables="{\"i\":{\"Probing\":\"ON\"},\"v\":{\"Probing\":\"ON\"}}"
  SPC{1..32} (32 alike) : nesl_utility/Simulink-PS Converter  PhysicalDomain=network_engine_domain  SubClassName=ps_input  LeftPortType=input  RightPortType=output  PseudoPeriodic=off  Frequencies=[]  NoiseDistribution=none  NoiseParameters=[]  Unit=1  AffineConversion=off  FilteringAndDerivatives=provide  SimscapeFilterOrder=1  InputFilterTimeConstant=0.001  UdotUserProvided=0
  SolverConfig : nesl_utility/Solver Configuration  PhysicalDomain=network_engine_domain  SubClassName=solver  LeftPortType=input  RightPortType=generic  Tones=[]  Harmonics=[]  SimulateNoise=off  Profile=off  UseLocalSampling=off  EnableSwitchedLinearOptims=on  FrequencyDomain=off  UseCCode=off  RelTol=0.001  AbsTol=0.001  MinStep=1e-09  ToWorkspace=off  RevertToSquareIcSolve=off  NumHomotopyIterations=100  PhasorMode=off  PhasorModeNumHarmonics=1  ConsistencySolver=NEWTON_XTOL_AFTER_FTOL  IndexReductionMethod=DerivativeReplacement  DoDC=off  ResidualTolerance=1e-09  ConsistencyTolSource=GLOBAL  ConsistencyAbsTol=0.001  ConsistencyRelTol=0.001  ConsistencyTolFactor=0.001  UseLocalSolver=off  LocalSolverChoice=NE_BACKWARD_EULER_ADVANCER  ResolveIndetEquations=on  FunctionEvalNumThread=1  LocalSolverSampleTime=0.001  DoFixedCost=off  MaxNonlinIter=3  MaxModeIter=2  ComputeImpulses=off  ImpulseIterations=2  LinearAlgebra=auto  LinearAlgebraNumThread=0  EquationFormulation=NE_TIME_EF  DelaysMemoryBudget=1024  AutomaticFiltering=on  FilteringTimeConstant=0.001  PartitionStorageMethod=AS_NEEDED  PartitionMemoryBudget=1024  PartitionMethod=ROBUST  MultibodyUseLocalSolver=off  MultibodyLocalSolverChoice=ODE1  MultibodyLocalSolverSampleTime=0.001
  TR_MA{1,5,9,13,17,21,25,29} (8 alike) : fl_lib/Thermal/Thermal Elements/Thermal Resistance  resistance=thermalResistanceModuleToAmbient_1 K/W  T_specify=off  T_priority=None  T=0 K  T_nominal_specify=off  T_nominal_value=1  T_nominal_unit=K  Q_specify=off  Q_priority=None  Q=0 W  Q_nominal_specify=off  Q_nominal_value=1  Q_nominal_unit=W
  TR_MA{2,6,10,14,18,22,26,30} (8 alike) : fl_lib/Thermal/Thermal Elements/Thermal Resistance  resistance=thermalResistanceModuleToAmbient_2 K/W  T_specify=off  T_priority=None  T=0 K  T_nominal_specify=off  T_nominal_value=1  T_nominal_unit=K  Q_specify=off  Q_priority=None  Q=0 W  Q_nominal_specify=off  Q_nominal_value=1  Q_nominal_unit=W
  TR_MA{3,7,11,15,19,23,27,31} (8 alike) : fl_lib/Thermal/Thermal Elements/Thermal Resistance  resistance=thermalResistanceModuleToAmbient_3 K/W  T_specify=off  T_priority=None  T=0 K  T_nominal_specify=off  T_nominal_value=1  T_nominal_unit=K  Q_specify=off  Q_priority=None  Q=0 W  Q_nominal_specify=off  Q_nominal_value=1  Q_nominal_unit=W
  TR_MA{4,8,12,16,20,24,28,32} (8 alike) : fl_lib/Thermal/Thermal Elements/Thermal Resistance  resistance=thermalResistanceModuleToAmbient_0 K/W  T_specify=off  T_priority=None  T=0 K  T_nominal_specify=off  T_nominal_value=1  T_nominal_unit=K  Q_specify=off  Q_priority=None  Q=0 W  Q_nominal_specify=off  Q_nominal_value=1  Q_nominal_unit=W
  TR_TMCPCC{1..32} (32 alike) : fl_lib/Thermal/Thermal Elements/Thermal Resistance  resistance=thermalResistanceTubeToModule K/W  T_specify=off  T_priority=None  T=0 K  T_nominal_specify=off  T_nominal_value=1  T_nominal_unit=K  Q_specify=off  Q_priority=None  Q=0 W  Q_nominal_specify=off  Q_nominal_value=1  Q_nominal_unit=W
  TR_TMCPHC{1..32} (32 alike) : fl_lib/Thermal/Thermal Elements/Thermal Resistance  resistance=thermalResistanceTubeToModule K/W  T_specify=off  T_priority=None  T=0 K  T_nominal_specify=off  T_nominal_value=1  T_nominal_unit=K  Q_specify=off  Q_priority=None  Q=0 W  Q_nominal_specify=off  Q_nominal_value=1  Q_nominal_unit=W
  TempProbeBlock1 : SimscapeProbe  BoundBlock=168  Variables="{\"M.T\":{\"Probing\":\"ON\"}}"
  TempProbeBlock10 : SimscapeProbe  BoundBlock=177  Variables="{\"M.T\":{\"Probing\":\"ON\"}}"
  TempProbeBlock11 : SimscapeProbe  BoundBlock=178  Variables="{\"M.T\":{\"Probing\":\"ON\"}}"
  TempProbeBlock12 : SimscapeProbe  BoundBlock=179  Variables="{\"M.T\":{\"Probing\":\"ON\"}}"
  TempProbeBlock13 : SimscapeProbe  BoundBlock=180  Variables="{\"M.T\":{\"Probing\":\"ON\"}}"
  TempProbeBlock14 : SimscapeProbe  BoundBlock=181  Variables="{\"M.T\":{\"Probing\":\"ON\"}}"
  TempProbeBlock15 : SimscapeProbe  BoundBlock=182  Variables="{\"M.T\":{\"Probing\":\"ON\"}}"
  TempProbeBlock16 : SimscapeProbe  BoundBlock=183  Variables="{\"M.T\":{\"Probing\":\"ON\"}}"
  TempProbeBlock17 : SimscapeProbe  BoundBlock=184  Variables="{\"M.T\":{\"Probing\":\"ON\"}}"
  TempProbeBlock18 : SimscapeProbe  BoundBlock=185  Variables="{\"M.T\":{\"Probing\":\"ON\"}}"
  TempProbeBlock19 : SimscapeProbe  BoundBlock=186  Variables="{\"M.T\":{\"Probing\":\"ON\"}}"
  TempProbeBlock2 : SimscapeProbe  BoundBlock=169  Variables="{\"M.T\":{\"Probing\":\"ON\"}}"
  TempProbeBlock20 : SimscapeProbe  BoundBlock=187  Variables="{\"M.T\":{\"Probing\":\"ON\"}}"
  TempProbeBlock21 : SimscapeProbe  BoundBlock=188  Variables="{\"M.T\":{\"Probing\":\"ON\"}}"
  TempProbeBlock22 : SimscapeProbe  BoundBlock=189  Variables="{\"M.T\":{\"Probing\":\"ON\"}}"
  TempProbeBlock23 : SimscapeProbe  BoundBlock=190  Variables="{\"M.T\":{\"Probing\":\"ON\"}}"
  TempProbeBlock24 : SimscapeProbe  BoundBlock=191  Variables="{\"M.T\":{\"Probing\":\"ON\"}}"
  TempProbeBlock25 : SimscapeProbe  BoundBlock=192  Variables="{\"M.T\":{\"Probing\":\"ON\"}}"
  TempProbeBlock26 : SimscapeProbe  BoundBlock=193  Variables="{\"M.T\":{\"Probing\":\"ON\"}}"
  TempProbeBlock27 : SimscapeProbe  BoundBlock=194  Variables="{\"M.T\":{\"Probing\":\"ON\"}}"
  TempProbeBlock28 : SimscapeProbe  BoundBlock=195  Variables="{\"M.T\":{\"Probing\":\"ON\"}}"
  TempProbeBlock29 : SimscapeProbe  BoundBlock=196  Variables="{\"M.T\":{\"Probing\":\"ON\"}}"
  TempProbeBlock3 : SimscapeProbe  BoundBlock=170  Variables="{\"M.T\":{\"Probing\":\"ON\"}}"
  TempProbeBlock30 : SimscapeProbe  BoundBlock=197  Variables="{\"M.T\":{\"Probing\":\"ON\"}}"
  TempProbeBlock31 : SimscapeProbe  BoundBlock=198  Variables="{\"M.T\":{\"Probing\":\"ON\"}}"
  TempProbeBlock32 : SimscapeProbe  BoundBlock=199  Variables="{\"M.T\":{\"Probing\":\"ON\"}}"
  TempProbeBlock4 : SimscapeProbe  BoundBlock=171  Variables="{\"M.T\":{\"Probing\":\"ON\"}}"
  TempProbeBlock5 : SimscapeProbe  BoundBlock=172  Variables="{\"M.T\":{\"Probing\":\"ON\"}}"
  TempProbeBlock6 : SimscapeProbe  BoundBlock=173  Variables="{\"M.T\":{\"Probing\":\"ON\"}}"
  TempProbeBlock7 : SimscapeProbe  BoundBlock=174  Variables="{\"M.T\":{\"Probing\":\"ON\"}}"
  TempProbeBlock8 : SimscapeProbe  BoundBlock=175  Variables="{\"M.T\":{\"Probing\":\"ON\"}}"
  TempProbeBlock9 : SimscapeProbe  BoundBlock=176  Variables="{\"M.T\":{\"Probing\":\"ON\"}}"
  TempSource : fl_lib/Thermal/Thermal Sources/Controlled Temperature Source
  ThermalMassBatteries{1..32} (32 alike) : fl_lib/Thermal/Thermal Elements/Thermal Mass  mass_type=foundation.enum.constant_variable.constant  mass=massModuleScale * scaledMassModule kg  sp_heat=CpModule J/(K*kg)  mass_min=1e-6 kg  num_ports=foundation.enum.numPorts2.one  m_specify=off  m_priority=High  m=1 kg  m_nominal_specify=off  m_nominal_value=1  m_nominal_unit=kg  T_specify=on  T_priority=High  T=AmbientTemperature K  T_nominal_specify=off  T_nominal_value=1  T_nominal_unit=K  Q_specify=off  Q_priority=None  Q=0 W  Q_nominal_specify=off  Q_nominal_value=1  Q_nominal_unit=W
  ThermalMassCPCC{1..32} (32 alike) : fl_lib/Thermal/Thermal Elements/Thermal Mass  mass_type=foundation.enum.constant_variable.constant  mass=massCoolantScale * scaledMassCoolant kg  sp_heat=CpCoolant J/(K*kg)  mass_min=1e-6 kg  num_ports=foundation.enum.numPorts2.one  m_specify=off  m_priority=High  m=1 kg  m_nominal_specify=off  m_nominal_value=1  m_nominal_unit=kg  T_specify=on  T_priority=High  T=AmbientTemperature K  T_nominal_specify=off  T_nominal_value=1  T_nominal_unit=K  Q_specify=off  Q_priority=None  Q=0 W  Q_nominal_specify=off  Q_nominal_value=1  Q_nominal_unit=W
  ThermalMassCPHC{1..32} (32 alike) : fl_lib/Thermal/Thermal Elements/Thermal Mass  mass_type=foundation.enum.constant_variable.constant  mass=massCoolantScale * scaledMassCoolant kg  sp_heat=CpCoolant J/(K*kg)  mass_min=1e-6 kg  num_ports=foundation.enum.numPorts2.one  m_specify=off  m_priority=High  m=1 kg  m_nominal_specify=off  m_nominal_value=1  m_nominal_unit=kg  T_specify=on  T_priority=High  T=AmbientTemperature K  T_nominal_specify=off  T_nominal_value=1  T_nominal_unit=K  Q_specify=off  Q_priority=None  Q=0 W  Q_nominal_specify=off  Q_nominal_value=1  Q_nominal_unit=W
  ThermalReference : fl_lib/Thermal/Thermal Elements/Thermal Reference
  ThermalReferenceInElectricalModel : fl_lib/Thermal/Thermal Elements/Thermal Reference
  ThermalSolverConfig : nesl_utility/Solver Configuration  PhysicalDomain=network_engine_domain  SubClassName=solver  LeftPortType=input  RightPortType=generic  Tones=[]  Harmonics=[]  SimulateNoise=off  Profile=off  UseLocalSampling=off  EnableSwitchedLinearOptims=on  FrequencyDomain=off  UseCCode=off  RelTol=0.001  AbsTol=0.001  MinStep=1e-09  ToWorkspace=off  RevertToSquareIcSolve=off  NumHomotopyIterations=100  PhasorMode=off  PhasorModeNumHarmonics=1  ConsistencySolver=NEWTON_XTOL_AFTER_FTOL  IndexReductionMethod=DerivativeReplacement  DoDC=off  ResidualTolerance=1e-09  ConsistencyTolSource=GLOBAL  ConsistencyAbsTol=0.001  ConsistencyRelTol=0.001  ConsistencyTolFactor=0.001  UseLocalSolver=off  LocalSolverChoice=NE_BACKWARD_EULER_ADVANCER  ResolveIndetEquations=on  FunctionEvalNumThread=1  LocalSolverSampleTime=0.001  DoFixedCost=off  MaxNonlinIter=3  MaxModeIter=2  ComputeImpulses=off  ImpulseIterations=2  LinearAlgebra=auto  LinearAlgebraNumThread=0  EquationFormulation=NE_TIME_EF  DelaysMemoryBudget=1024  AutomaticFiltering=on  FilteringTimeConstant=0.001  PartitionStorageMethod=AS_NEEDED  PartitionMemoryBudget=1024  PartitionMethod=ROBUST  MultibodyUseLocalSolver=off  MultibodyLocalSolverChoice=ODE1  MultibodyLocalSolverSampleTime=0.001
  coolantSwitch : coolantFlowSwitch_lib/MATLAB Function  SystemSampleTime=-1  VariantActivationTime=update diagram  EmptyChoice=off  PassThrough=off  PassThroughVariantControl=(default)  EmptyChoiceVariantControl=(default)  AllowFlexibleInterface=on  Latency=0  AutoFrameSizeCalculation=off
  coolantSwitchConverter : nesl_utility/Simulink-PS Converter  PhysicalDomain=network_engine_domain  SubClassName=ps_input  LeftPortType=input  RightPortType=output  PseudoPeriodic=off  Frequencies=[]  NoiseDistribution=none  NoiseParameters=[]  Unit=1  AffineConversion=off  FilteringAndDerivatives=provide  SimscapeFilterOrder=1  InputFilterTimeConstant=0.001  UdotUserProvided=0
  coolantSwitchMultiplier : fl_lib/Physical Signals/Functions/PS Product
  currentProfiletoSimscape : nesl_utility/Simulink-PS Converter  PhysicalDomain=network_engine_domain  SubClassName=ps_input  LeftPortType=input  RightPortType=output  PseudoPeriodic=off  Frequencies=[]  NoiseDistribution=none  NoiseParameters=[]  Unit=1  AffineConversion=off  FilteringAndDerivatives=provide  SimscapeFilterOrder=1  InputFilterTimeConstant=0.001  UdotUserProvided=0
  heat{1..32} (32 alike) : fl_lib/Thermal/Thermal Sources/Controlled Heat Flow Rate Source
  heatGenModule{1..32} (32 alike) : heatGenerationForCellResolvedModel/heatGenCellResolved  SystemSampleTime=-1  VariantActivationTime=update diagram  EmptyChoice=off  PassThrough=off  PassThroughVariantControl=(default)  EmptyChoiceVariantControl=(default)  AllowFlexibleInterface=on  Latency=0  AutoFrameSizeCalculation=off
  tempSource{1..32} (32 alike) : fl_lib/Thermal/Thermal Sources/Controlled Temperature Source
  thermalToElectricalConverter{1..32} (32 alike) : nesl_utility/Simulink-PS Converter  PhysicalDomain=network_engine_domain  SubClassName=ps_input  LeftPortType=input  RightPortType=output  PseudoPeriodic=off  Frequencies=[]  NoiseDistribution=none  NoiseParameters=[]  Unit=K  AffineConversion=off  FilteringAndDerivatives=filter  SimscapeFilterOrder=1  InputFilterTimeConstant=0.001  UdotUserProvided=0
  Conn1 : PMIOPort  Side=Left
  Out1 : Outport
  Out2 : Outport  Port=2
  wires:
  heatGenModule13/1 -> SPC13/1
  heatGenModule14/1 -> SPC14/1
  heatGenModule11/1 -> SPC11/1
  heatGenModule16/1 -> SPC16/1
  MyProbeBlock11/4 -> heatGenModule11/4
  heatGenModule18/1 -> SPC18/1
  TempProbeBlock13/1 -> thermalToElectricalConverter13/1  "T13"
  TempProbeBlock10/1 -> thermalToElectricalConverter10/1  "T10"
  TempProbeBlock26/1 -> thermalToElectricalConverter26/1  "T26"
  TempProbeBlock25/1 -> thermalToElectricalConverter25/1  "T25"
  TempProbeBlock28/1 -> thermalToElectricalConverter28/1  "T28"
  TempProbeBlock30/1 -> thermalToElectricalConverter30/1  "T30"
  TempProbeBlock32/1 -> thermalToElectricalConverter32/1  "T32"
  MyProbeBlock26/4 -> heatGenModule26/4
  MyProbeBlock26/2 -> heatGenModule26/2
  MyProbeBlock18/3 -> heatGenModule18/3
  heatGenModule24/1 -> SPC24/1
  MyProbeBlock25/4 -> heatGenModule25/4
  TempProbeBlock29/1 -> thermalToElectricalConverter29/1  "T29"
  heatGenModule7/1 -> SPC7/1
  MyProbeBlock32/2 -> heatGenModule32/2
  MyProbeBlock23/3 -> heatGenModule23/3
  MyProbeBlock27/1 -> heatGenModule27/1
  MyProbeBlock5/2 -> heatGenModule5/2
  heatGenModule15/1 -> SPC15/1
  heatGenModule17/1 -> SPC17/1
  MyProbeBlock3/4 -> heatGenModule3/4
  MyProbeBlock32/3 -> heatGenModule32/3
  MyProbeBlock8/1 -> heatGenModule8/1
  MyProbeBlock15/2 -> heatGenModule15/2
  MyProbeBlock21/4 -> heatGenModule21/4
  MyProbeBlock17/2 -> heatGenModule17/2
  MyProbeBlock21/1 -> heatGenModule21/1
  MyProbeBlock7/3 -> heatGenModule7/3
  MyProbeBlock17/3 -> heatGenModule17/3
  TempProbeBlock7/1 -> thermalToElectricalConverter7/1  "T7"
  MyProbeBlock24/4 -> heatGenModule24/4
  MyProbeBlock14/2 -> heatGenModule14/2
  MyProbeBlock13/3 -> heatGenModule13/3
  heatGenModule6/1 -> SPC6/1
  MyProbeBlock16/2 -> heatGenModule16/2
  MyProbeBlock3/1 -> heatGenModule3/1
  MyProbeBlock13/4 -> heatGenModule13/4
  MyProbeBlock7/4 -> heatGenModule7/4
  MyProbeBlock20/2 -> heatGenModule20/2
  MyProbeBlock19/4 -> heatGenModule19/4
  MyProbeBlock27/3 -> heatGenModule27/3
  MyProbeBlock6/2 -> heatGenModule6/2
  MyProbeBlock9/2 -> heatGenModule9/2
  MyProbeBlock6/4 -> heatGenModule6/4
  MyProbeBlock28/2 -> heatGenModule28/2
  MyProbeBlock13/1 -> heatGenModule13/1
  MyProbeBlock8/4 -> heatGenModule8/4
  MyProbeBlock10/2 -> heatGenModule10/2
  MyProbeBlock23/2 -> heatGenModule23/2
  heatGenModule21/1 -> SPC21/1
  MyProbeBlock26/1 -> heatGenModule26/1
  MyProbeBlock7/2 -> heatGenModule7/2
  MyProbeBlock5/1 -> heatGenModule5/1
  heatGenModule31/1 -> SPC31/1
  MyProbeBlock12/2 -> heatGenModule12/2
  MyProbeBlock4/2 -> heatGenModule4/2
  heatGenModule19/1 -> SPC19/1
  MyProbeBlock4/3 -> heatGenModule4/3
  heatGenModule30/1 -> SPC30/1
  heatGenModule9/1 -> SPC9/1
  MyProbeBlock25/3 -> heatGenModule25/3
  heatGenModule10/1 -> SPC10/1
  MyProbeBlock17/1 -> heatGenModule17/1
  MyProbeBlock3/2 -> heatGenModule3/2
  MyProbeBlock5/4 -> heatGenModule5/4
  MyProbeBlock2/3 -> heatGenModule2/3
  MyProbeBlock24/3 -> heatGenModule24/3
  heatGenModule25/1 -> SPC25/1
  MyProbeBlock2/4 -> heatGenModule2/4
  TempProbeBlock20/1 -> thermalToElectricalConverter20/1  "T20"
  heatGenModule1/1 -> SPC1/1
  MyProbeBlock9/3 -> heatGenModule9/3
  MyProbeBlock13/2 -> heatGenModule13/2
  heatGenModule26/1 -> SPC26/1
  TempProbeBlock5/1 -> thermalToElectricalConverter5/1  "T5"
  MyProbeBlock19/3 -> heatGenModule19/3
  TempProbeBlock22/1 -> thermalToElectricalConverter22/1  "T22"
  TempProbeBlock31/1 -> thermalToElectricalConverter31/1  "T31"
  heatGenModule3/1 -> SPC3/1
  TempProbeBlock16/1 -> thermalToElectricalConverter16/1  "T16"
  MyProbeBlock29/4 -> heatGenModule29/4
  MyProbeBlock6/1 -> heatGenModule6/1
  MyProbeBlock14/4 -> heatGenModule14/4
  heatGenModule8/1 -> SPC8/1
  MyProbeBlock32/1 -> heatGenModule32/1
  MyProbeBlock20/4 -> heatGenModule20/4
  MyProbeBlock15/4 -> heatGenModule15/4
  TempProbeBlock27/1 -> thermalToElectricalConverter27/1  "T27"
  MyProbeBlock9/1 -> heatGenModule9/1
  TempProbeBlock3/1 -> thermalToElectricalConverter3/1  "T3"
  MyProbeBlock1/1 -> heatGenModule1/1
  MyProbeBlock15/3 -> heatGenModule15/3
  heatGenModule22/1 -> SPC22/1
  MyProbeBlock12/4 -> heatGenModule12/4
  MyProbeBlock18/4 -> heatGenModule18/4
  heatGenModule23/1 -> SPC23/1
  MyProbeBlock2/1 -> heatGenModule2/1
  MyProbeBlock31/3 -> heatGenModule31/3
  MyProbeBlock23/1 -> heatGenModule23/1
  PackProbe/2 -> Out2/1
  MyProbeBlock5/3 -> heatGenModule5/3
  MyProbeBlock31/2 -> heatGenModule31/2
  heatGenModule28/1 -> SPC28/1
  MyProbeBlock28/3 -> heatGenModule28/3
  MyProbeBlock30/1 -> heatGenModule30/1
  MyProbeBlock8/3 -> heatGenModule8/3
  TempProbeBlock24/1 -> thermalToElectricalConverter24/1  "T24"
  MyProbeBlock14/1 -> heatGenModule14/1
  MyProbeBlock15/1 -> heatGenModule15/1
  MyProbeBlock29/2 -> heatGenModule29/2
  PackProbe/1 -> Out1/1
  MyProbeBlock16/1 -> heatGenModule16/1
  MyProbeBlock11/1 -> heatGenModule11/1
  MyProbeBlock6/3 -> heatGenModule6/3
  MyProbeBlock23/4 -> heatGenModule23/4
  MyProbeBlock31/1 -> heatGenModule31/1
  MyProbeBlock8/2 -> heatGenModule8/2
  MyProbeBlock19/1 -> heatGenModule19/1
  MyProbeBlock11/2 -> heatGenModule11/2
  MyProbeBlock11/3 -> heatGenModule11/3
  TempProbeBlock21/1 -> thermalToElectricalConverter21/1  "T21"
  MyProbeBlock30/3 -> heatGenModule30/3
  heatGenModule5/1 -> SPC5/1
  MyProbeBlock12/1 -> heatGenModule12/1
  MyProbeBlock4/1 -> heatGenModule4/1
  MyProbeBlock24/2 -> heatGenModule24/2
  MyProbeBlock29/1 -> heatGenModule29/1
  MyProbeBlock7/1 -> heatGenModule7/1
  input0/1 -> currentProfiletoSimscape/1, coolantSwitch/1
  MyProbeBlock2/2 -> heatGenModule2/2
  MyProbeBlock19/2 -> heatGenModule19/2
  MyProbeBlock20/3 -> heatGenModule20/3
  MyProbeBlock16/4 -> heatGenModule16/4
  MyProbeBlock28/1 -> heatGenModule28/1
  MyProbeBlock27/4 -> heatGenModule27/4
  MyProbeBlock32/4 -> heatGenModule32/4
  TempProbeBlock4/1 -> thermalToElectricalConverter4/1  "T4"
  MyProbeBlock24/1 -> heatGenModule24/1
  TempProbeBlock12/1 -> thermalToElectricalConverter12/1  "T12"
